simulink model "SwarmSystem"  (R2022b)
(part 3 of 4)

\"uuid\":\"66f2432a-d8da-4c77-847a-13be9309f023\"},{\"content\":{\"blockPath\":[\"SwarmSystem/Record\"],\"channel\":[7,2,1],\"dimensions\":[9,9,3],\"domain\":\"SwarmSystem/Record\",\"lineColor\":\"#ff6929\",\"parentID\":5326,\"plots\":[],\"port\":9,\"sid\":[\"\"],\"signalID\":5732,\"signalName\":\"packed_tw\"},\"type\":\"RecordBlkView.Signal\",\"uuid\":\"56f2028f-166f-4731-ad48-c59b44126da3\"},{\"content\":{\"blockPath\":[\"SwarmSystem/Record\"],\"channel\":[8,2,1],\"dimensions\":[9,9,3],\"domain\":\"SwarmSystem/Record\",\"lineColor\":\"#b746ff\",\"parentID\":5326,\"plots\":[],\"port\":9,\"sid\":[\"\"],\"signalID\":5733,\"signalName\":\"packed_tw\"},\"type\":\"RecordBlkView.Signal\",\"uuid\":\"6663be21-9b2e-46ef-97ca-d0d1a511769f\"},{\"content\":{\"blockPath\":[\"SwarmSystem/Record\"],\"channel\":[9,2,1],\"dimensions\":[9,9,3],\"domain\":\"SwarmSystem/Record\",\"lineColor\":\"#64d413\",\"parentID\":5326,\"plots\":[],\"port\":9,\"sid\":[\"\"],\"signalID\":5734,\"signalName\":\"packed_tw\"},\"type\":\"RecordBlkView.Signal\",\"uuid\":\"2c203f91-17b3-4c19-9696-d99f0a1ca0fd\"},{\"content\":{\"blockPath\":[\"SwarmSystem/Record\"],\"channel\":[1,3,1],\"dimensions\":[9,9,3],\"domain\":\"SwarmSystem/Record\",\"lineColor\":\"#ff13a6\",\"parentID\":5326,\"plots\":[],\"port\":9,\"sid\":[\"\"],\"signalID\":5735,\"signalName\":\"packed_tw\"},\"type\":\"RecordBlkView.Signal\",\"uuid\":\"a7da77ac-4730-4896-99b2-25e0e7a6f8af\"},{\"content\":{\"blockPath\":[\"SwarmSystem/Record\"],\"channel\":[2,3,1],\"dimensions\":[9,9,3],\"domain\":\"SwarmSystem/Record\",\"lineColor\":\"#fe330a\",\"parentID\":5326,\"plots\":[],\"port\":9,\"sid\":[\"\"],\"signalID\":5736,\"signalName\":\"packed_tw\"},\"type\":\"RecordBlkView.Signal\",\"uuid\":\"1e600a43-36ad-42ac-b351-5715d6370cc7\"},{\"content\":{\"blockPath\":[\"SwarmSystem/Record\"],\"channel\":[3,3,1],\"dimensions\":[9,9,3],\"domain\":\"SwarmSystem/Record\",\"lineColor\":\"#22b573\",\"parentID\":5326,\"plots\":[],\"port\":9,\"sid\":[\"\"],\"signalID\":5737,\"signalName\":\"packed_tw\"},\"type\":\"RecordBlkView.Signal\",\"uuid\":\"10fccabd-f891-426d-aafe-525a94df6eca\"},{\"content\":{\"blockPath\":[\"SwarmSystem/Record\"],\"channel\":[4,3,1],\"dimensions\":[9,9,3],\"domain\":\"SwarmSystem/Record\",\"lineColor\":\"#0072bd\",\"parentID\":5326,\"plots\":[],\"port\":9,\"sid\":[\"\"],\"signalID\":5738,\"signalName\":\"packed_tw\"},\"type\":\"RecordBlkView.Signal\",\"uuid\":\"d8f853b9-8d61-485c-b86b-01323a9b1dcc\"},{\"content\":{\"blockPath\":[\"SwarmSystem/Record\"],\"channel\":[5,3,1],\"dimensions\":[9,9,3],\"domain\":\"SwarmSystem/Record\",\"lineColor\":\"#d95319\",\"parentID\":5326,\"plots\":[],\"port\":9,\"sid\":[\"\"],\"signalID\":5739,\"signalName\":\"packed_tw\"},\"type\":\"RecordBlkView.Signal\",\"uuid\":\"32f64f79-0b5d-41ec-b8f2-db72d15c3b46\"},{\"content\":{\"blockPath\":[\"SwarmSystem/Record\"],\"channel\":[6,3,1],\"dimensions\":[9,9,3],\"domain\":\"SwarmSystem/Record\",\"lineColor\":\"#edb120\",\"parentID\":5326,\"plots\":[],\"port\":9,\"sid\":[\"\"],\"signalID\":5740,\"signalName\":\"packed_tw\"},\"type\":\"RecordBlkView.Signal\",\"uuid\":\"6bb0f485-e50d-4674-9966-5c0abecf3566\"},{\"content\":{\"blockPath\":[\"SwarmSystem/Record\"],\"channel\":[7,3,1],\"dimensions\":[9,9,3],\"domain\":\"SwarmSystem/Record\",\"lineColor\":\"#7e2f8e\",\"parentID\":5326,\"plots\":[],\"port\":9,\"sid\":[\"\"],\"signalID\":5741,\"signalName\":\"packed_tw\"},\"type\":\"RecordBlkView.Signal\",\"uuid\":\"efdbdfa0-ad42-48dc-a3e2-49e98de60d36\"},{\"content\":{\"blockPath\":[\"SwarmSystem/Record\"],\"channel\":[8,3,1],\"dimensions\":[9,9,3],\"domain\":\"SwarmSystem/Record\",\"lineColor\":\"#77ac30\",\"parentID\":5326,\"plots\":[],\"port\":9,\"sid\":[\"\"],\"signalID\":5742,\"signalName\":\"packed_tw\"},\"type\":\"RecordBlkView.Signal\",\"uuid\":\"b0fc06d3-33ee-41bb-9294-d6c8533c9df3\"},{\"content\":{\"blockPath\":[\"SwarmSystem/Record\"],\"channel\":[9,3,1],\"dimensions\":[9,9,3],\"domain\":\"SwarmSystem/Record\",\"lineColor\":\"#4dbeee\",\"parentID\":5326,\"plots\":[],\"port\":9,\"sid\":[\"\"],\"signalID\":5743,\"signalName\":\"packed_tw\"},\"type\":\"RecordBlkView.Signal\",\"uuid\":\"376f8440-522b-4ce7-8b3c-728053a193f3\"},{\"content\":{\"blockPath\":[\"SwarmSystem/Record\"],\"channel\":[1,4,1],\"dimensions\":[9,9,3],\"domain\":\"SwarmSystem/Record\",\"lineColor\":\"#a2142f\",\"parentID\":5326,\"plots\":[],\"port\":9,\"sid\":[\"\"],\"signalID\":5744,\"signalName\":\"packed_tw\"},\"type\":\"RecordBlkView.Signal\",\"uuid\":\"16833fa1-bc7e-4160-bf2a-8aa71fa237a6\"},{\"content\":{\"blockPath\":[\"SwarmSystem/Record\"],\"channel\":[2,4,1],\"dimensions\":[9,9,3],\"domain\":\"SwarmSystem/Record\",\"lineColor\":\"#139fff\",\"parentID\":5326,\"plots\":[],\"port\":9,\"sid\":[\"\"],\"signalID\":5745,\"signalName\":\"packed_tw\"},\"type\":\"RecordBlkView.Signal\",\"uuid\":\"0f9268d8-1260-481f-958d-5a37cc72ea48\"},{\"content\":{\"blockPath\":[\"SwarmSystem/Record\"],\"channel\":[3,4,1],\"dimensions\":[9,9,3],\"domain\":\"SwarmSystem/Record\",\"lineColor\":\"#ff6929\",\"parentID\":5326,\"plots\":[],\"port\":9,\"sid\":[\"\"],\"signalID\":5746,\"signalName\":\"packed_tw\"},\"type\":\"RecordBlkView.Signal\",\"uuid\":\"582107cd-b22c-4bf8-875e-6a25fbec9bc4\"},{\"content\":{\"blockPath\":[\"SwarmSystem/Record\"],\"channel\":[4,4,1],\"dimensions\":[9,9,3],\"domain\":\"SwarmSystem/Record\",\"lineColor\":\"#b746ff\",\"parentID\":5326,\"plots\":[],\"port\":9,\"sid\":[\"\"],\"signalID\":5747,\"signalName\":\"packed_tw\"},\"type\":\"RecordBlkView.Signal\",\"uuid\":\"86fb42d5-9bfb-4257-8da5-ea0cdfb8f8a8\"},{\"content\":{\"blockPath\":[\"SwarmSystem/Record\"],\"channel\":[5,4,1],\"dimensions\":[9,9,3],\"domain\":\"SwarmSystem/Record\",\"lineColor\":\"#64d413\",\"parentID\":5326,\"plots\":[],\"port\":9,\"sid\":[\"\"],\"signalID\":5748,\"signalName\":\"packed_tw\"},\"type\":\"RecordBlkView.Signal\",\"uuid\":\"152469c8-5e3d-42f9-b5e4-54b25046ce6a\"},{\"content\":{\"blockPath\":[\"SwarmSystem/Record\"],\"channel\":[6,4,1],\"dimensions\":[9,9,3],\"domain\":\"SwarmSystem/Record\",\"lineColor\":\"#ff13a6\",\"parentID\":5326,\"plots\":[],\"port\":9,\"sid\":[\"\"],\"signalID\":5749,\"signalName\":\"packed_tw\"},\"type\":\"RecordBlkView.Signal\",\"uuid\":\"f025a8fe-ae08-4e09-9d36-edd1af49b1c7\"},{\"content\":{\"blockPath\":[\"SwarmSystem/Record\"],\"channel\":[7,4,1],\"dimensions\":[9,9,3],\"domain\":\"SwarmSystem/Record\",\"lineColor\":\"#fe330a\",\"parentID\":5326,\"plots\":[],\"port\":9,\"sid\":[\"\"],\"signalID\":5750,\"signalName\":\"packed_tw\"},\"type\":\"RecordBlkView.Signal\",\"uuid\":\"d6d3dd3c-ecca-4921-b9f8-a246ee4cded9\"},{\"content\":{\"blockPath\":[\"SwarmSystem/Record\"],\"channel\":[8,4,1],\"dimensions\":[9,9,3],\"domain\":\"SwarmSystem/Record\",\"lineColor\":\"#22b573\",\"parentID\":5326,\"plots\":[],\"port\":9,\"sid\":[\"\"],\"signalID\":5751,\"signalName\":\"packed_tw\"},\"type\":\"RecordBlkView.Signal\",\"uuid\":\"cb92334f-db7b-47eb-97a9-d6af63c7032c\"},{\"content\":{\"blockPath\":[\"SwarmSystem/Record\"],\"channel\":[9,4,1],\"dimensions\":[9,9,3],\"domain\":\"SwarmSystem/Record\",\"lineColor\":\"#0072bd\",\"parentID\":5326,\"plots\":[],\"port\":9,\"sid\":[\"\"],\"signalID\":5752,\"signalName\":\"packed_tw\"},\"type\":\"RecordBlkView.Signal\",\"uuid\":\"410ffef6-764f-4449-b289-13b898e3b605\"},{\"content\":{\"blockPath\":[\"SwarmSystem/Record\"],\"channel\":[1,5,1],\"dimensions\":[9,9,3],\"domain\":\"SwarmSystem/Record\",\"lineColor\":\"#d95319\",\"parentID\":5326,\"plots\":[],\"port\":9,\"sid\":[\"\"],\"signalID\":5753,\"signalName\":\"packed_tw\"},\"type\":\"RecordBlkView.Signal\",\"uuid\":\"e261075f-568b-4d5f-8c86-3e293640aaf6\"},{\"content\":{\"blockPath\":[\"SwarmSystem/Record\"],\"channel\":[2,5,1],\"dimensions\":[9,9,3],\"domain\":\"SwarmSystem/Record\",\"lineColor\":\"#edb120\",\"parentID\":5326,\"plots\":[],\"port\":9,\"sid\":[\"\"],\"signalID\":5754,\"signalName\":\"packed_tw\"},\"type\":\"RecordBlkView.Signal\",\"uuid\":\"02d9d080-5992-4875-a7e4-490970fd0aba\"},{\"content\":{\"blockPath\":[\"SwarmSystem/Record\"],\"channel\":[3,5,1],\"dimensions\":[9,9,3],\"domain\":\"SwarmSystem/Record\",\"lineColor\":\"#7e2f8e\",\"parentID\":5326,\"plots\":[],\"port\":9,\"sid\":[\"\"],\"signalID\":5755,\"signalName\":\"packed_tw\"},\"type\":\"RecordBlkView.Signal\",\"uuid\":\"f6234f5e-dfa5-4099-ab9d-213a77899b41\"},{\"content\":{\"blockPath\":[\"SwarmSystem/Record\"],\"channel\":[4,5,1],\"dimensions\":[9,9,3],\"domain\":\"SwarmSystem/Record\",\"lineColor\":\"#77ac30\",\"parentID\":5326,\"plots\":[],\"port\":9,\"sid\":[\"\"],\"signalID\":5756,\"signalName\":\"packed_tw\"},\"type\":\"RecordBlkView.Signal\",\"uuid\":\"897adc16-ad91-416a-abb4-75db18956903\"},{\"content\":{\"blockPath\":[\"SwarmSystem/Record\"],\"channel\":[5,5,1],\"dimensions\":[9,9,3],\"domain\":\"SwarmSystem/Record\",\"lineColor\":\"#4dbeee\",\"parentID\":5326,\"plots\":[],\"port\":9,\"sid\":[\"\"],\"signalID\":5757,\"signalName\":\"packed_tw\"},\"type\":\"RecordBlkView.Signal\",\"uuid\":\"0cc5aa6a-a08c-40bc-a91d-690ed3804433\"},{\"content\":{\"blockPath\":[\"SwarmSystem/Record\"],\"channel\":[6,5,1],\"dimensions\":[9,9,3],\"domain\":\"SwarmSystem/Record\",\"lineColor\":\"#a2142f\",\"parentID\":5326,\"plots\":[],\"port\":9,\"sid\":[\"\"],\"signalID\":5758,\"signalName\":\"packed_tw\"},\"type\":\"RecordBlkView.Signal\",\"uuid\":\"667ed152-3318-44bb-b581-6255efbc3158\"},{\"content\":{\"blockPath\":[\"SwarmSystem/Record\"],\"channel\":[7,5,1],\"dimensions\":[9,9,3],\"domain\":\"SwarmSystem/Record\",\"lineColor\":\"#139fff\",\"parentID\":5326,\"plots\":[],\"port\":9,\"sid\":[\"\"],\"signalID\":5759,\"signalName\":\"packed_tw\"},\"type\":\"RecordBlkView.Signal\",\"uuid\":\"c45443c0-bb0f-43ce-ae46-f6908f651d0a\"},{\"content\":{\"blockPath\":[\"SwarmSystem/Record\"],\"channel\":[8,5,1],\"dimensions\":[9,9,3],\"domain\":\"SwarmSystem/Record\",\"lineColor\":\"#ff6929\",\"parentID\":5326,\"plots\":[],\"port\":9,\"sid\":[\"\"],\"signalID\":5760,\"signalName\":\"packed_tw\"},\"type\":\"RecordBlkView.Signal\",\"uuid\":\"3b7accaa-1a50-42c4-810c-86a74667a25e\"},{\"content\":{\"blockPath\":[\"SwarmSystem/Record\"],\"channel\":[9,5,1],\"dimensions\":[9,9,3],\"domain\":\"SwarmSystem/Record\",\"lineColor\":\"#b746ff\",\"parentID\":5326,\"plots\":[],\"port\":9,\"sid\":[\"\"],\"signalID\":5761,\"signalName\":\"packed_tw\"},\"type\":\"RecordBlkView.Signal\",\"uuid\":\"4a9e9fa2-2054-41d9-b7b8-434b94a0f53e\"},{\"content\":{\"blockPath\":[\"SwarmSystem/Record\"],\"channel\":[1,6,1],\"dimensions\":[9,9,3],\"domain\":\"SwarmSystem/Record\",\"lineColor\":\"#64d413\",\"parentID\":5326,\"plots\":[],\"port\":9,\"sid\":[\"\"],\"signalID\":5762,\"signalName\":\"packed_tw\"},\"type\":\"RecordBlkView.Signal\",\"uuid\":\"2f297c1c-5db3-4597-bca3-5568c9b68469\"},{\"content\":{\"blockPath\":[\"SwarmSystem/Record\"],\"channel\":[2,6,1],\"dimensions\":[9,9,3],\"domain\":\"SwarmSystem/Record\",\"lineColor\":\"#ff13a6\",\"parentID\":5326,\"plots\":[],\"port\":9,\"sid\":[\"\"],\"signalID\":5763,\"signalName\":\"packed_tw\"},\"type\":\"RecordBlkView.Signal\",\"uuid\":\"3bcefa39-97a0-4915-bf31-1d3eb75403ff\"},{\"content\":{\"blockPath\":[\"SwarmSystem/Record\"],\"channel\":[3,6,1],\"dimensions\":[9,9,3],\"domain\":\"SwarmSystem/Record\",\"lineColor\":\"#fe330a\",\"parentID\":5326,\"plots\":[],\"port\":9,\"sid\":[\"\"],\"signalID\":5764,\"signalName\":\"packed_tw\"},\"type\":\"RecordBlkView.Signal\",\"uuid\":\"26a823e5-a67c-4fe0-8814-e404e1866f34\"},{\"content\":{\"blockPath\":[\"SwarmSystem/Record\"],\"channel\":[4,6,1],\"dimensions\":[9,9,3],\"domain\":\"SwarmSystem/Record\",\"lineColor\":\"#22b573\",\"parentID\":5326,\"plots\":[],\"port\":9,\"sid\":[\"\"],\"signalID\":5765,\"signalName\":\"packed_tw\"},\"type\":\"RecordBlkView.Signal\",\"uuid\":\"0219ef0b-387c-40a0-97df-a2f3b60856a0\"},{\"content\":{\"blockPath\":[\"SwarmSystem/Record\"],\"channel\":[5,6,1],\"dimensions\":[9,9,3],\"domain\":\"SwarmSystem/Record\",\"lineColor\":\"#0072bd\",\"parentID\":5326,\"plots\":[],\"port\":9,\"sid\":[\"\"],\"signalID\":5766,\"signalName\":\"packed_tw\"},\"type\":\"RecordBlkView.Signal\",\"uuid\":\"e0fe79da-d3e3-475c-af43-7a4fae6dd308\"},{\"content\":{\"blockPath\":[\"SwarmSystem/Record\"],\"channel\":[6,6,1],\"dimensions\":[9,9,3],\"domain\":\"SwarmSystem/Record\",\"lineColor\":\"#d95319\",\"parentID\":5326,\"plots\":[],\"port\":9,\"sid\":[\"\"],\"signalID\":5767,\"signalName\":\"packed_tw\"},\"type\":\"RecordBlkView.Signal\",\"uuid\":\"25247346-aef6-4321-9915-4b5ba2b68a3c\"},{\"content\":{\"blockPath\":[\"SwarmSystem/Record\"],\"channel\":[7,6,1],\"dimensions\":[9,9,3],\"domain\":\"SwarmSystem/Record\",\"lineColor\":\"#edb120\",\"parentID\":5326,\"plots\":[],\"port\":9,\"sid\":[\"\"],\"signalID\":5768,\"signalName\":\"packed_tw\"},\"type\":\"RecordBlkView.Signal\",\"uuid\":\"d5d8b9f2-a0d1-4825-ac7f-db45dff184b1\"},{\"content\":{\"blockPath\":[\"SwarmSystem/Record\"],\"channel\":[8,6,1],\"dimensions\":[9,9,3],\"domain\":\"SwarmSystem/Record\",\"lineColor\":\"#7e2f8e\",\"parentID\":5326,\"plots\":[],\"port\":9,\"sid\":[\"\"],\"signalID\":5769,\"signalName\":\"packed_tw\"},\"type\":\"RecordBlkView.Signal\",\"uuid\":\"c3c3fecf-6756-4264-a6b3-b17d8feaae56\"},{\"content\":{\"blockPath\":[\"SwarmSystem/Record\"],\"channel\":[9,6,1],\"dimensions\":[9,9,3],\"domain\":\"SwarmSystem/Record\",\"lineColor\":\"#77ac30\",\"parentID\":5326,\"plots\":[],\"port\":9,\"sid\":[\"\"],\"signalID\":5770,\"signalName\":\"packed_tw\"},\"type\":\"RecordBlkView.Signal\",\"uuid\":\"95d6af73-0c27-4f58-aa73-e4afb520c9b6\"},{\"content\":{\"blockPath\":[\"SwarmSystem/Record\"],\"channel\":[1,7,1],\"dimensions\":[9,9,3],\"domain\":\"SwarmSystem/Record\",\"lineColor\":\"#4dbeee\",\"parentID\":5326,\"plots\":[],\"port\":9,\"sid\":[\"\"],\"signalID\":5771,\"signalName\":\"packed_tw\"},\"type\":\"RecordBlkView.Signal\",\"uuid\":\"ffa40b6e-c93c-45e7-a825-7543730c02a7\"},{\"content\":{\"blockPath\":[\"SwarmSystem/Record\"],\"channel\":[2,7,1],\"dimensions\":[9,9,3],\"domain\":\"SwarmSystem/Record\",\"lineColor\":\"#a2142f\",\"parentID\":5326,\"plots\":[],\"port\":9,\"sid\":[\"\"],\"signalID\":5772,\"signalName\":\"packed_tw\"},\"type\":\"RecordBlkView.Signal\",\"uuid\":\"572a2db8-4bea-405f-acfc-7af25e433108\"},{\"content\":{\"blockPath\":[\"SwarmSystem/Record\"],\"channel\":[3,7,1],\"dimensions\":[9,9,3],\"domain\":\"SwarmSystem/Record\",\"lineColor\":\"#139fff\",\"parentID\":5326,\"plots\":[],\"port\":9,\"sid\":[\"\"],\"signalID\":5773,\"signalName\":\"packed_tw\"},\"type\":\"RecordBlkView.Signal\",\"uuid\":\"0dfc27a1-e3b2-4639-b1fe-a522ef6232c5\"},{\"content\":{\"blockPath\":[\"SwarmSystem/Record\"],\"channel\":[4,7,1],\"dimensions\":[9,9,3],\"domain\":\"SwarmSystem/Record\",\"lineColor\":\"#ff6929\",\"parentID\":5326,\"plots\":[],\"port\":9,\"sid\":[\"\"],\"signalID\":5774,\"signalName\":\"packed_tw\"},\"type\":\"RecordBlkView.Signal\",\"uuid\":\"6f7742b4-e30b-4d3b-9c5b-bb79d8c25ffc\"},{\"content\":{\"blockPath\":[\"SwarmSystem/Record\"],\"channel\":[5,7,1],\"dimensions\":[9,9,3],\"domain\":\"SwarmSystem/Record\",\"lineColor\":\"#b746ff\",\"parentID\":5326,\"plots\":[],\"port\":9,\"sid\":[\"\"],\"signalID\":5775,\"signalName\":\"packed_tw\"},\"type\":\"RecordBlkView.Signal\",\"uuid\":\"1bed10ed-21c7-4778-9f87-780cf6804573\"},{\"content\":{\"blockPath\":[\"SwarmSystem/Record\"],\"channel\":[6,7,1],\"dimensions\":[9,9,3],\"domain\":\"SwarmSystem/Record\",\"lineColor\":\"#64d413\",\"parentID\":5326,\"plots\":[],\"port\":9,\"sid\":[\"\"],\"signalID\":5776,\"signalName\":\"packed_tw\"},\"type\":\"RecordBlkView.Signal\",\"uuid\":\"f026d189-9db8-4d86-976b-f51f0daa1cbb\"},{\"content\":{\"blockPath\":[\"SwarmSystem/Record\"],\"channel\":[7,7,1],\"dimensions\":[9,9,3],\"domain\":\"SwarmSystem/Record\",\"lineColor\":\"#ff13a6\",\"parentID\":5326,\"plots\":[],\"port\":9,\"sid\":[\"\"],\"signalID\":5777,\"signalName\":\"packed_tw\"},\"type\":\"RecordBlkView.Signal\",\"uuid\":\"693525ca-a567-456e-a572-dbfb87322e0c\"},{\"content\":{\"blockPath\":[\"SwarmSystem/Record\"],\"channel\":[8,7,1],\"dimensions\":[9,9,3],\"domain\":\"SwarmSystem/Record\",\"lineColor\":\"#fe330a\",\"parentID\":5326,\"plots\":[],\"port\":9,\"sid\":[\"\"],\"signalID\":5778,\"signalName\":\"packed_tw\"},\"type\":\"RecordBlkView.Signal\",\"uuid\":\"67c23147-ccbd-4398-b187-1940e8bea18b\"},{\"content\":{\"blockPath\":[\"SwarmSystem/Record\"],\"channel\":[9,7,1],\"dimensions\":[9,9,3],\"domain\":\"SwarmSystem/Record\",\"lineColor\":\"#22b573\",\"parentID\":5326,\"plots\":[],\"port\":9,\"sid\":[\"\"],\"signalID\":5779,\"signalName\":\"packed_tw\"},\"type\":\"RecordBlkView.Signal\",\"uuid\":\"97770466-2798-420b-969b-754700610d6d\"},{\"content\":{\"blockPath\":[\"SwarmSystem/Record\"],\"channel\":[1,8,1],\"dimensions\":[9,9,3],\"domain\":\"SwarmSystem/Record\",\"lineColor\":\"#0072bd\",\"parentID\":5326,\"plots\":[],\"port\":9,\"sid\":[\"\"],\"signalID\":5780,\"signalName\":\"packed_tw\"},\"type\":\"RecordBlkView.Signal\",\"uuid\":\"c0d727bd-d530-42f1-bdd3-579b10f7c70f\"},{\"content\":{\"blockPath\":[\"SwarmSystem/Record\"],\"channel\":[2,8,1],\"dimensions\":[9,9,3],\"domain\":\"SwarmSystem/Record\",\"lineColor\":\"#d95319\",\"parentID\":5326,\"plots\":[],\"port\":9,\"sid\":[\"\"],\"signalID\":5781,\"signalName\":\"packed_tw\"},\"type\":\"RecordBlkView.Signal\",\"uuid\":\"e95a2d2e-be99-4a14-8ecc-e91ebfb0d15f\"},{\"content\":{\"blockPath\":[\"SwarmSystem/Record\"],\"channel\":[3,8,1],\"dimensions\":[9,9,3],\"domain\":\"SwarmSystem/Record\",\"lineColor\":\"#edb120\",\"parentID\":5326,\"plots\":[],\"port\":9,\"sid\":[\"\"],\"signalID\":5782,\"signalName\":\"packed_tw\"},\"type\":\"RecordBlkView.Signal\",\"uuid\":\"618e1a82-3965-4102-97cc-7656c92e492e\"},{\"content\":{\"blockPath\":[\"SwarmSystem/Record\"],\"channel\":[4,8,1],\"dimensions\":[9,9,3],\"domain\":\"SwarmSystem/Record\",\"lineColor\":\"#7e2f8e\",\"parentID\":5326,\"plots\":[],\"port\":9,\"sid\":[\"\"],\"signalID\":5783,\"signalName\":\"packed_tw\"},\"type\":\"RecordBlkView.Signal\",\"uuid\":\"5a512c5a-af72-415b-bdc8-3aa69033ccbb\"},{\"content\":{\"blockPath\":[\"SwarmSystem/Record\"],\"channel\":[5,8,1],\"dimensions\":[9,9,3],\"domain\":\"SwarmSystem/Record\",\"lineColor\":\"#77ac30\",\"parentID\":5326,\"plots\":[],\"port\":9,\"sid\":[\"\"],\"signalID\":5784,\"signalName\":\"packed_tw\"},\"type\":\"RecordBlkView.Signal\",\"uuid\":\"e955dfcf-7950-4eba-bd26-624af6308b70\"},{\"content\":{\"blockPath\":[\"SwarmSystem/Record\"],\"channel\":[6,8,1],\"dimensions\":[9,9,3],\"domain\":\"SwarmSystem/Record\",\"lineColor\":\"#4dbeee\",\"parentID\":5326,\"plots\":[],\"port\":9,\"sid\":[\"\"],\"signalID\":5785,\"signalName\":\"packed_tw\"},\"type\":\"RecordBlkView.Signal\",\"uuid\":\"ece48233-0de4-42a5-9ae6-f029001ff023\"},{\"content\":{\"blockPath\":[\"SwarmSystem/Record\"],\"channel\":[7,8,1],\"dimensions\":[9,9,3],\"domain\":\"SwarmSystem/Record\",\"lineColor\":\"#a2142f\",\"parentID\":5326,\"plots\":[],\"port\":9,\"sid\":[\"\"],\"signalID\":5786,\"signalName\":\"packed_tw\"},\"type\":\"RecordBlkView.Signal\",\"uuid\":\"824bdf22-e070-493b-b58d-fb5a60069d4e\"},{\"content\":{\"blockPath\":[\"SwarmSystem/Record\"],\"channel\":[8,8,1],\"dimensions\":[9,9,3],\"domain\":\"SwarmSystem/Record\",\"lineColor\":\"#139fff\",\"parentID\":5326,\"plots\":[],\"port\":9,\"sid\":[\"\"],\"signalID\":5787,\"signalName\":\"packed_tw\"},\"type\":\"RecordBlkView.Signal\",\"uuid\":\"caa1d600-3dac-4235-a1df-80f1f38b6da0\"},{\"content\":{\"blockPath\":[\"SwarmSystem/Record\"],\"channel\":[9,8,1],\"dimensions\":[9,9,3],\"domain\":\"SwarmSystem/Record\",\"lineColor\":\"#ff6929\",\"parentID\":5326,\"plots\":[],\"port\":9,\"sid\":[\"\"],\"signalID\":5788,\"signalName\":\"packed_tw\"},\"type\":\"RecordBlkView.Signal\",\"uuid\":\"70268a07-477f-46a3-bb7c-da2b62262bc9\"},{\"content\":{\"blockPath\":[\"SwarmSystem/Record\"],\"channel\":[1,9,1],\"dimensions\":[9,9,3],\"domain\":\"SwarmSystem/Record\",\"lineColor\":\"#b746ff\",\"parentID\":5326,\"plots\":[],\"port\":9,\"sid\":[\"\"],\"signalID\":5789,\"signalName\":\"packed_tw\"},\"type\":\"RecordBlkView.Signal\",\"uuid\":\"d68f7306-5943-43c0-978b-d9ecc93acb51\"},{\"content\":{\"blockPath\":[\"SwarmSystem/Record\"],\"channel\":[2,9,1],\"dimensions\":[9,9,3],\"domain\":\"SwarmSystem/Record\",\"lineColor\":\"#64d413\",\"parentID\":5326,\"plots\":[],\"port\":9,\"sid\":[\"\"],\"signalID\":5790,\"signalName\":\"packed_tw\"},\"type\":\"RecordBlkView.Signal\",\"uuid\":\"edf609c4-3d89-44f9-9262-dda908b0e004\"},{\"content\":{\"blockPath\":[\"SwarmSystem/Record\"],\"channel\":[3,9,1],\"dimensions\":[9,9,3],\"domain\":\"SwarmSystem/Record\",\"lineColor\":\"#ff13a6\",\"parentID\":5326,\"plots\":[],\"port\":9,\"sid\":[\"\"],\"signalID\":5791,\"signalName\":\"packed_tw\"},\"type\":\"RecordBlkView.Signal\",\"uuid\":\"1f514293-d0a4-426d-8fe5-839bc86e8e90\"},{\"content\":{\"blockPath\":[\"SwarmSystem/Record\"],\"channel\":[4,9,1],\"dimensions\":[9,9,3],\"domain\":\"SwarmSystem/Record\",\"lineColor\":\"#fe330a\",\"parentID\":5326,\"plots\":[],\"port\":9,\"sid\":[\"\"],\"signalID\":5792,\"signalName\":\"packed_tw\"},\"type\":\"RecordBlkView.Signal\",\"uuid\":\"9ed22710-5236-4372-8da5-48d9aff1790b\"},{\"content\":{\"blockPath\":[\"SwarmSystem/Record\"],\"channel\":[5,9,1],\"dimensions\":[9,9,3],\"domain\":\"SwarmSystem/Record\",\"lineColor\":\"#22b573\",\"parentID\":5326,\"plots\":[],\"port\":9,\"sid\":[\"\"],\"signalID\":5793,\"signalName\":\"packed_tw\"},\"type\":\"RecordBlkView.Signal\",\"uuid\":\"31fcf3e9-d45c-439a-97b6-eb5fde562b10\"},{\"content\":{\"blockPath\":[\"SwarmSystem/Record\"],\"channel\":[6,9,1],\"dimensions\":[9,9,3],\"domain\":\"SwarmSystem/Record\",\"lineColor\":\"#0072bd\",\"parentID\":5326,\"plots\":[],\"port\":9,\"sid\":[\"\"],\"signalID\":5794,\"signalName\":\"packed_tw\"},\"type\":\"RecordBlkView.Signal\",\"uuid\":\"9bcc6742-29be-48e2-89c3-fd54e1edf038\"},{\"content\":{\"blockPath\":[\"SwarmSystem/Record\"],\"channel\":[7,9,1],\"dimensions\":[9,9,3],\"domain\":\"SwarmSystem/Record\",\"lineColor\":\"#d95319\",\"parentID\":5326,\"plots\":[],\"port\":9,\"sid\":[\"\"],\"signalID\":5795,\"signalName\":\"packed_tw\"},\"type\":\"RecordBlkView.Signal\",\"uuid\":\"961200f8-714d-4018-af6a-2f1112332411\"},{\"content\":{\"blockPath\":[\"SwarmSystem/Record\"],\"channel\":[8,9,1],\"dimensions\":[9,9,3],\"domain\":\"SwarmSystem/Record\",\"lineColor\":\"#edb120\",\"parentID\":5326,\"plots\":[],\"port\":9,\"sid\":[\"\"],\"signalID\":5796,\"signalName\":\"packed_tw\"},\"type\":\"RecordBlkView.Signal\",\"uuid\":\"c1ea7ad4-a570-4cc9-90b0-014c375aaef8\"},{\"content\":{\"blockPath\":[\"SwarmSystem/Record\"],\"channel\":[9,9,1],\"dimensions\":[9,9,3],\"domain\":\"SwarmSystem/Record\",\"lineColor\":\"#7e2f8e\",\"parentID\":5326,\"plots\":[],\"port\":9,\"sid\":[\"\"],\"signalID\":5797,\"signalName\":\"packed_tw\"},\"type\":\"RecordBlkView.Signal\",\"uuid\":\"cb727bd5-f244-448c-a21d-edf04e397600\"},{\"content\":{\"blockPath\":[\"SwarmSystem/Record\"],\"channel\":[1,1,2],\"dimensions\":[9,9,3],\"domain\":\"SwarmSystem/Record\",\"lineColor\":\"#77ac30\",\"parentID\":5326,\"plots\":[],\"port\":9,\"sid\":[\"\"],\"signalID\":5798,\"signalName\":\"packed_tw\"},\"type\":\"RecordBlkView.Signal\",\"uuid\":\"cb38d9e5-ffd7-459c-8e44-38c3f8cd33c6\"},{\"content\":{\"blockPath\":[\"SwarmSystem/Record\"],\"channel\":[2,1,2],\"dimensions\":[9,9,3],\"domain\":\"SwarmSystem/Record\",\"lineColor\":\"#4dbeee\",\"parentID\":5326,\"plots\":[],\"port\":9,\"sid\":[\"\"],\"signalID\":5799,\"signalName\":\"packed_tw\"},\"type\":\"RecordBlkView.Signal\",\"uuid\":\"25e48605-b9a0-4eff-9681-4ea1dedc7113\"},{\"content\":{\"blockPath\":[\"SwarmSystem/Record\"],\"channel\":[3,1,2],\"dimensions\":[9,9,3],\"domain\":\"SwarmSystem/Record\",\"lineColor\":\"#a2142f\",\"parentID\":5326,\"plots\":[],\"port\":9,\"sid\":[\"\"],\"signalID\":5800,\"signalName\":\"packed_tw\"},\"type\":\"RecordBlkView.Signal\",\"uuid\":\"46ac54a4-10b4-4c2f-a611-f8be5c9883b4\"},{\"content\":{\"blockPath\":[\"SwarmSystem/Record\"],\"channel\":[4,1,2],\"dimensions\":[9,9,3],\"domain\":\"SwarmSystem/Record\",\"lineColor\":\"#139fff\",\"parentID\":5326,\"plots\":[],\"port\":9,\"sid\":[\"\"],\"signalID\":5801,\"signalName\":\"packed_tw\"},\"type\":\"RecordBlkView.Signal\",\"uuid\":\"ac218199-2d6d-4ea5-a8c1-aacdddd33c28\"},{\"content\":{\"blockPath\":[\"SwarmSystem/Record\"],\"channel\":[5,1,2],\"dimensions\":[9,9,3],\"domain\":\"SwarmSystem/Record\",\"lineColor\":\"#ff6929\",\"parentID\":5326,\"plots\":[],\"port\":9,\"sid\":[\"\"],\"signalID\":5802,\"signalName\":\"packed_tw\"},\"type\":\"RecordBlkView.Signal\",\"uuid\":\"f55d1ba3-9854-45c1-8251-dd3b01695bb6\"},{\"content\":{\"blockPath\":[\"SwarmSystem/Record\"],\"channel\":[6,1,2],\"dimensions\":[9,9,3],\"domain\":\"SwarmSystem/Record\",\"lineColor\":\"#b746ff\",\"parentID\":5326,\"plots\":[],\"port\":9,\"sid\":[\"\"],\"signalID\":5803,\"signalName\":\"packed_tw\"},\"type\":\"RecordBlkView.Signal\",\"uuid\":\"024d7ef1-8905-4559-97f9-831c79e47f0f\"},{\"content\":{\"blockPath\":[\"SwarmSystem/Record\"],\"channel\":[7,1,2],\"dimensions\":[9,9,3],\"domain\":\"SwarmSystem/Record\",\"lineColor\":\"#64d413\",\"parentID\":5326,\"plots\":[],\"port\":9,\"sid\":[\"\"],\"signalID\":5804,\"signalName\":\"packed_tw\"},\"type\":\"RecordBlkView.Signal\",\"uuid\":\"8ccd5203-03c3-4fcd-94b7-203d27d26910\"},{\"content\":{\"blockPath\":[\"SwarmSystem/Record\"],\"channel\":[8,1,2],\"dimensions\":[9,9,3],\"domain\":\"SwarmSystem/Record\",\"lineColor\":\"#ff13a6\",\"parentID\":5326,\"plots\":[],\"port\":9,\"sid\":[\"\"],\"signalID\":5805,\"signalName\":\"packed_tw\"},\"type\":\"RecordBlkView.Signal\",\"uuid\":\"6dd5faa0-5582-4c32-84a6-9e6d74d4ab74\"},{\"content\":{\"blockPath\":[\"SwarmSystem/Record\"],\"channel\":[9,1,2],\"dimensions\":[9,9,3],\"domain\":\"SwarmSystem/Record\",\"lineColor\":\"#fe330a\",\"parentID\":5326,\"plots\":[],\"port\":9,\"sid\":[\"\"],\"signalID\":5806,\"signalName\":\"packed_tw\"},\"type\":\"RecordBlkView.Signal\",\"uuid\":\"effa1f6f-5389-411d-88e5-57b121372908\"},{\"content\":{\"blockPath\":[\"SwarmSystem/Record\"],\"channel\":[1,2,2],\"dimensions\":[9,9,3],\"domain\":\"SwarmSystem/Record\",\"lineColor\":\"#22b573\",\"parentID\":5326,\"plots\":[],\"port\":9,\"sid\":[\"\"],\"signalID\":5807,\"signalName\":\"packed_tw\"},\"type\":\"RecordBlkView.Signal\",\"uuid\":\"60e694a9-3551-482f-9541-9e908d86fb43\"},{\"content\":{\"blockPath\":[\"SwarmSystem/Record\"],\"channel\":[2,2,2],\"dimensions\":[9,9,3],\"domain\":\"SwarmSystem/Record\",\"lineColor\":\"#0072bd\",\"parentID\":5326,\"plots\":[],\"port\":9,\"sid\":[\"\"],\"signalID\":5808,\"signalName\":\"packed_tw\"},\"type\":\"RecordBlkView.Signal\",\"uuid\":\"64585b29-3283-4af9-89d1-c59c492422c2\"},{\"content\":{\"blockPath\":[\"SwarmSystem/Record\"],\"channel\":[3,2,2],\"dimensions\":[9,9,3],\"domain\":\"SwarmSystem/Record\",\"lineColor\":\"#d95319\",\"parentID\":5326,\"plots\":[],\"port\":9,\"sid\":[\"\"],\"signalID\":5809,\"signalName\":\"packed_tw\"},\"type\":\"RecordBlkView.Signal\",\"uuid\":\"e1f20fe9-1db5-4066-87d6-318fe0e498e9\"},{\"content\":{\"blockPath\":[\"SwarmSystem/Record\"],\"channel\":[4,2,2],\"dimensions\":[9,9,3],\"domain\":\"SwarmSystem/Record\",\"lineColor\":\"#edb120\",\"parentID\":5326,\"plots\":[],\"port\":9,\"sid\":[\"\"],\"signalID\":5810,\"signalName\":\"packed_tw\"},\"type\":\"RecordBlkView.Signal\",\"uuid\":\"930acee9-4257-4c9a-99a8-349e59c5c7d9\"},{\"content\":{\"blockPath\":[\"SwarmSystem/Record\"],\"channel\":[5,2,2],\"dimensions\":[9,9,3],\"domain\":\"SwarmSystem/Record\",\"lineColor\":\"#7e2f8e\",\"parentID\":5326,\"plots\":[],\"port\":9,\"sid\":[\"\"],\"signalID\":5811,\"signalName\":\"packed_tw\"},\"type\":\"RecordBlkView.Signal\",\"uuid\":\"42f198cf-b7e2-45a5-8eec-73d355926375\"},{\"content\":{\"blockPath\":[\"SwarmSystem/Record\"],\"channel\":[6,2,2],\"dimensions\":[9,9,3],\"domain\":\"SwarmSystem/Record\",\"lineColor\":\"#77ac30\",\"parentID\":5326,\"plots\":[],\"port\":9,\"sid\":[\"\"],\"signalID\":5812,\"signalName\":\"packed_tw\"},\"type\":\"RecordBlkView.Signal\",\"uuid\":\"af41296c-0c3d-45c8-a859-59d45e13e9c2\"},{\"content\":{\"blockPath\":[\"SwarmSystem/Record\"],\"channel\":[7,2,2],\"dimensions\":[9,9,3],\"domain\":\"SwarmSystem/Record\",\"lineColor\":\"#4dbeee\",\"parentID\":5326,\"plots\":[],\"port\":9,\"sid\":[\"\"],\"signalID\":5813,\"signalName\":\"packed_tw\"},\"type\":\"RecordBlkView.Signal\",\"uuid\":\"e673c85c-3b38-4b09-a889-1e246211c421\"},{\"content\":{\"blockPath\":[\"SwarmSystem/Record\"],\"channel\":[8,2,2],\"dimensions\":[9,9,3],\"domain\":\"SwarmSystem/Record\",\"lineColor\":\"#a2142f\",\"parentID\":5326,\"plots\":[],\"port\":9,\"sid\":[\"\"],\"signalID\":5814,\"signalName\":\"packed_tw\"},\"type\":\"RecordBlkView.Signal\",\"uuid\":\"0ef2cfa8-3698-4975-baf2-f02ae27c6b5c\"},{\"content\":{\"blockPath\":[\"SwarmSystem/Record\"],\"channel\":[9,2,2],\"dimensions\":[9,9,3],\"domain\":\"SwarmSystem/Record\",\"lineColor\":\"#139fff\",\"parentID\":5326,\"plots\":[],\"port\":9,\"sid\":[\"\"],\"signalID\":5815,\"signalName\":\"packed_tw\"},\"type\":\"RecordBlkView.Signal\",\"uuid\":\"2c305bdd-f00d-47e3-a104-3da68df50175\"},{\"content\":{\"blockPath\":[\"SwarmSystem/Record\"],\"channel\":[1,3,2],\"dimensions\":[9,9,3],\"domain\":\"SwarmSystem/Record\",\"lineColor\":\"#ff6929\",\"parentID\":5326,\"plots\":[],\"port\":9,\"sid\":[\"\"],\"signalID\":5816,\"signalName\":\"packed_tw\"},\"type\":\"RecordBlkView.Signal\",\"uuid\":\"553ce6f2-2ed6-40c5-a20e-983dfc431183\"},{\"content\":{\"blockPath\":[\"SwarmSystem/Record\"],\"channel\":[2,3,2],\"dimensions\":[9,9,3],\"domain\":\"SwarmSystem/Record\",\"lineColor\":\"#b746ff\",\"parentID\":5326,\"plots\":[],\"port\":9,\"sid\":[\"\"],\"signalID\":5817,\"signalName\":\"packed_tw\"},\"type\":\"RecordBlkView.Signal\",\"uuid\":\"89f353a5-7a81-461b-a22e-736f12088d8e\"},{\"content\":{\"blockPath\":[\"SwarmSystem/Record\"],\"channel\":[3,3,2],\"dimensions\":[9,9,3],\"domain\":\"SwarmSystem/Record\",\"lineColor\":\"#64d413\",\"parentID\":5326,\"plots\":[],\"port\":9,\"sid\":[\"\"],\"signalID\":5818,\"signalName\":\"packed_tw\"},\"type\":\"RecordBlkView.Signal\",\"uuid\":\"9c8ba869-9418-4a08-8767-18862245c084\"},{\"content\":{\"blockPath\":[\"SwarmSystem/Record\"],\"channel\":[4,3,2],\"dimensions\":[9,9,3],\"domain\":\"SwarmSystem/Record\",\"lineColor\":\"#ff13a6\",\"parentID\":5326,\"plots\":[],\"port\":9,\"sid\":[\"\"],\"signalID\":5819,\"signalName\":\"packed_tw\"},\"type\":\"RecordBlkView.Signal\",\"uuid\":\"c861881c-da11-4fd0-b8fb-73a7150c480e\"},{\"content\":{\"blockPath\":[\"SwarmSystem/Record\"],\"channel\":[5,3,2],\"dimensions\":[9,9,3],\"domain\":\"SwarmSystem/Record\",\"lineColor\":\"#fe330a\",\"parentID\":5326,\"plots\":[],\"port\":9,\"sid\":[\"\"],\"signalID\":5820,\"signalName\":\"packed_tw\"},\"type\":\"RecordBlkView.Signal\",\"uuid\":\"c9f9dad2-6c58-4512-ba52-96053e8c0cac\"},{\"content\":{\"blockPath\":[\"SwarmSystem/Record\"],\"channel\":[6,3,2],\"dimensions\":[9,9,3],\"domain\":\"SwarmSystem/Record\",\"lineColor\":\"#22b573\",\"parentID\":5326,\"plots\":[],\"port\":9,\"sid\":[\"\"],\"signalID\":5821,\"signalName\":\"packed_tw\"},\"type\":\"RecordBlkView.Signal\",\"uuid\":\"316f2dc2-43f8-48d7-88b4-a124a1a2146f\"},{\"content\":{\"blockPath\":[\"SwarmSystem/Record\"],\"channel\":[7,3,2],\"dimensions\":[9,9,3],\"domain\":\"SwarmSystem/Record\",\"lineColor\":\"#0072bd\",\"parentID\":5326,\"plots\":[],\"port\":9,\"sid\":[\"\"],\"signalID\":5822,\"signalName\":\"packed_tw\"},\"type\":\"RecordBlkView.Signal\",\"uuid\":\"00eb1436-1d6d-4b52-8758-987c3d3c700f\"},{\"content\":{\"blockPath\":[\"SwarmSystem/Record\"],\"channel\":[8,3,2],\"dimensions\":[9,9,3],\"domain\":\"SwarmSystem/Record\",\"lineColor\":\"#d95319\",\"parentID\":5326,\"plots\":[],\"port\":9,\"sid\":[\"\"],\"signalID\":5823,\"signalName\":\"packed_tw\"},\"type\":\"RecordBlkView.Signal\",\"uuid\":\"ab7e27e8-5321-4674-ba25-1205592251f9\"},{\"content\":{\"blockPath\":[\"SwarmSystem/Record\"],\"channel\":[9,3,2],\"dimensions\":[9,9,3],\"domain\":\"SwarmSystem/Record\",\"lineColor\":\"#edb120\",\"parentID\":5326,\"plots\":[],\"port\":9,\"sid\":[\"\"],\"signalID\":5824,\"signalName\":\"packed_tw\"},\"type\":\"RecordBlkView.Signal\",\"uuid\":\"d9834565-c616-4685-982e-2acf66321c2f\"},{\"content\":{\"blockPath\":[\"SwarmSystem/Record\"],\"channel\":[1,4,2],\"dimensions\":[9,9,3],\"domain\":\"SwarmSystem/Record\",\"lineColor\":\"#7e2f8e\",\"parentID\":5326,\"plots\":[],\"port\":9,\"sid\":[\"\"],\"signalID\":5825,\"signalName\":\"packed_tw\"},\"type\":\"RecordBlkView.Signal\",\"uuid\":\"73a8f051-ac54-418b-be34-57c1bea9c926\"},{\"content\":{\"blockPath\":[\"SwarmSystem/Record\"],\"channel\":[2,4,2],\"dimensions\":[9,9,3],\"domain\":\"SwarmSystem/Record\",\"lineColor\":\"#77ac30\",\"parentID\":5326,\"plots\":[],\"port\":9,\"sid\":[\"\"],\"signalID\":5826,\"signalName\":\"packed_tw\"},\"type\":\"RecordBlkView.Signal\",\"uuid\":\"ec901a96-64ba-450d-8db8-9e10e434bb41\"},{\"content\":{\"blockPath\":[\"SwarmSystem/Record\"],\"channel\":[3,4,2],\"dimensions\":[9,9,3],\"domain\":\"SwarmSystem/Record\",\"lineColor\":\"#4dbeee\",\"parentID\":5326,\"plots\":[],\"port\":9,\"sid\":[\"\"],\"signalID\":5827,\"signalName\":\"packed_tw\"},\"type\":\"RecordBlkView.Signal\",\"uuid\":\"534b9c5f-68be-4bd8-b4a6-75f5e7942e28\"},{\"content\":{\"blockPath\":[\"SwarmSystem/Record\"],\"channel\":[4,4,2],\"dimensions\":[9,9,3],\"domain\":\"SwarmSystem/Record\",\"lineColor\":\"#a2142f\",\"parentID\":5326,\"plots\":[],\"port\":9,\"sid\":[\"\"],\"signalID\":5828,\"signalName\":\"packed_tw\"},\"type\":\"RecordBlkView.Signal\",\"uuid\":\"57cb10d4-3295-407a-b4d9-6c20fce866fa\"},{\"content\":{\"blockPath\":[\"SwarmSystem/Record\"],\"channel\":[5,4,2],\"dimensions\":[9,9,3],\"domain\":\"SwarmSystem/Record\",\"lineColor\":\"#139fff\",\"parentID\":5326,\"plots\":[],\"port\":9,\"sid\":[\"\"],\"signalID\":5829,\"signalName\":\"packed_tw\"},\"type\":\"RecordBlkView.Signal\",\"uuid\":\"f5f3c6c1-4e62-4e43-b99f-60b52f41186b\"},{\"content\":{\"blockPath\":[\"SwarmSystem/Record\"],\"channel\":[6,4,2],\"dimensions\":[9,9,3],\"domain\":\"SwarmSystem/Record\",\"lineColor\":\"#ff6929\",\"parentID\":5326,\"plots\":[],\"port\":9,\"sid\":[\"\"],\"signalID\":5830,\"signalName\":\"packed_tw\"},\"type\":\"RecordBlkView.Signal\",\"uuid\":\"dc35dde6-03e7-4e6f-96f1-92d578fc4cc8\"},{\"content\":{\"blockPath\":[\"SwarmSystem/Record\"],\"channel\":[7,4,2],\"dimensions\":[9,9,3],\"domain\":\"SwarmSystem/Record\",\"lineColor\":\"#b746ff\",\"parentID\":5326,\"plots\":[],\"port\":9,\"sid\":[\"\"],\"signalID\":5831,\"signalName\":\"packed_tw\"},\"type\":\"RecordBlkView.Signal\",\"uuid\":\"fb50e130-57ac-4c05-99f1-ad9b0756c040\"},{\"content\":{\"blockPath\":[\"SwarmSystem/Record\"],\"channel\":[8,4,2],\"dimensions\":[9,9,3],\"domain\":\"SwarmSystem/Record\",\"lineColor\":\"#64d413\",\"parentID\":5326,\"plots\":[],\"port\":9,\"sid\":[\"\"],\"signalID\":5832,\"signalName\":\"packed_tw\"},\"type\":\"RecordBlkView.Signal\",\"uuid\":\"dba0bcf1-9b0a-48a3-aae0-fa7dbe3bde5c\"},{\"content\":{\"blockPath\":[\"SwarmSystem/Record\"],\"channel\":[9,4,2],\"dimensions\":[9,9,3],\"domain\":\"SwarmSystem/Record\",\"lineColor\":\"#ff13a6\",\"parentID\":5326,\"plots\":[],\"port\":9,\"sid\":[\"\"],\"signalID\":5833,\"signalName\":\"packed_tw\"},\"type\":\"RecordBlkView.Signal\",\"uuid\":\"1cebf3f3-22dc-42d8-be53-d17a558b4ebc\"},{\"content\":{\"blockPath\":[\"SwarmSystem/Record\"],\"channel\":[1,5,2],\"dimensions\":[9,9,3],\"domain\":\"SwarmSystem/Record\",\"lineColor\":\"#fe330a\",\"parentID\":5326,\"plots\":[],\"port\":9,\"sid\":[\"\"],\"signalID\":5834,\"signalName\":\"packed_tw\"},\"type\":\"RecordBlkView.Signal\",\"uuid\":\"4fa55bca-6c09-4e46-a298-f94e0ea4cde9\"},{\"content\":{\"blockPath\":[\"SwarmSystem/Record\"],\"channel\":[2,5,2],\"dimensions\":[9,9,3],\"domain\":\"SwarmSystem/Record\",\"lineColor\":\"#22b573\",\"parentID\":5326,\"plots\":[],\"port\":9,\"sid\":[\"\"],\"signalID\":5835,\"signalName\":\"packed_tw\"},\"type\":\"RecordBlkView.Signal\",\"uuid\":\"d9747375-d0b0-44d0-95bb-be2acc7336b4\"},{\"content\":{\"blockPath\":[\"SwarmSystem/Record\"],\"channel\":[3,5,2],\"dimensions\":[9,9,3],\"domain\":\"SwarmSystem/Record\",\"lineColor\":\"#0072bd\",\"parentID\":5326,\"plots\":[],\"port\":9,\"sid\":[\"\"],\"signalID\":5836,\"signalName\":\"packed_tw\"},\"type\":\"RecordBlkView.Signal\",\"uuid\":\"8fc234f2-8d4e-4730-aa50-051c53edd537\"},{\"content\":{\"blockPath\":[\"SwarmSystem/Record\"],\"channel\":[4,5,2],\"dimensions\":[9,9,3],\"domain\":\"SwarmSystem/Record\",\"lineColor\":\"#d95319\",\"parentID\":5326,\"plots\":[],\"port\":9,\"sid\":[\"\"],\"signalID\":5837,\"signalName\":\"packed_tw\"},\"type\":\"RecordBlkView.Signal\",\"uuid\":\"a560e1ad-7774-4d9f-84bb-5f05b7e7085f\"},{\"content\":{\"blockPath\":[\"SwarmSystem/Record\"],\"channel\":[5,5,2],\"dimensions\":[9,9,3],\"domain\":\"SwarmSystem/Record\",\"lineColor\":\"#edb120\",\"parentID\":5326,\"plots\":[],\"port\":9,\"sid\":[\"\"],\"signalID\":5838,\"signalName\":\"packed_tw\"},\"type\":\"RecordBlkView.Signal\",\"uuid\":\"fd6ffdc4-27b6-4286-a4fe-fc74007b7de1\"},{\"content\":{\"blockPath\":[\"SwarmSystem/Record\"],\"channel\":[6,5,2],\"dimensions\":[9,9,3],\"domain\":\"SwarmSystem/Record\",\"lineColor\":\"#7e2f8e\",\"parentID\":5326,\"plots\":[],\"port\":9,\"sid\":[\"\"],\"signalID\":5839,\"signalName\":\"packed_tw\"},\"type\":\"RecordBlkView.Signal\",\"uuid\":\"30fe91e8-e058-4076-8567-0aa02a5d7a8b\"},{\"content\":{\"blockPath\":[\"SwarmSystem/Record\"],\"channel\":[7,5,2],\"dimensions\":[9,9,3],\"domain\":\"SwarmSystem/Record\",\"lineColor\":\"#77ac30\",\"parentID\":5326,\"plots\":[],\"port\":9,\"sid\":[\"\"],\"signalID\":5840,\"signalName\":\"packed_tw\"},\"type\":\"RecordBlkView.Signal\",\"uuid\":\"4d8de427-c42c-47e2-9661-72de3c01d0ec\"},{\"content\":{\"blockPath\":[\"SwarmSystem/Record\"],\"channel\":[8,5,2],\"dimensions\":[9,9,3],\"domain\":\"SwarmSystem/Record\",\"lineColor\":\"#4dbeee\",\"parentID\":5326,\"plots\":[],\"port\":9,\"sid\":[\"\"],\"signalID\":5841,\"signalName\":\"packed_tw\"},\"type\":\"RecordBlkView.Signal\",\"uuid\":\"74cb2627-61cd-403d-a7f2-2a0ab0ef8735\"},{\"content\":{\"blockPath\":[\"SwarmSystem/Record\"],\"channel\":[9,5,2],\"dimensions\":[9,9,3],\"domain\":\"SwarmSystem/Record\",\"lineColor\":\"#a2142f\",\"parentID\":5326,\"plots\":[],\"port\":9,\"sid\":[\"\"],\"signalID\":5842,\"signalName\":\"packed_tw\"},\"type\":\"RecordBlkView.Signal\",\"uuid\":\"afaaa2ce-30f7-42df-9fa7-b477d412027f\"},{\"content\":{\"blockPath\":[\"SwarmSystem/Record\"],\"channel\":[1,6,2],\"dimensions\":[9,9,3],\"domain\":\"SwarmSystem/Record\",\"lineColor\":\"#139fff\",\"parentID\":5326,\"plots\":[],\"port\":9,\"sid\":[\"\"],\"signalID\":5843,\"signalName\":\"packed_tw\"},\"type\":\"RecordBlkView.Signal\",\"uuid\":\"2b9b8baf-bf8c-43d3-8545-d5dd11e917b6\"},{\"content\":{\"blockPath\":[\"SwarmSystem/Record\"],\"channel\":[2,6,2],\"dimensions\":[9,9,3],\"domain\":\"SwarmSystem/Record\",\"lineColor\":\"#ff6929\",\"parentID\":5326,\"plots\":[],\"port\":9,\"sid\":[\"\"],\"signalID\":5844,\"signalName\":\"packed_tw\"},\"type\":\"RecordBlkView.Signal\",\"uuid\":\"27da3e74-6207-4525-b469-5e6bde21a3cc\"},{\"content\":{\"blockPath\":[\"SwarmSystem/Record\"],\"channel\":[3,6,2],\"dimensions\":[9,9,3],\"domain\":\"SwarmSystem/Record\",\"lineColor\":\"#b746ff\",\"parentID\":5326,\"plots\":[],\"port\":9,\"sid\":[\"\"],\"signalID\":5845,\"signalName\":\"packed_tw\"},\"type\":\"RecordBlkView.Signal\",\"uuid\":\"ec549dc2-6e7b-4aa4-8717-32341151da85\"},{\"content\":{\"blockPath\":[\"SwarmSystem/Record\"],\"channel\":[4,6,2],\"dimensions\":[9,9,3],\"domain\":\"SwarmSystem/Record\",\"lineColor\":\"#64d413\",\"parentID\":5326,\"plots\":[],\"port\":9,\"sid\":[\"\"],\"signalID\":5846,\"signalName\":\"packed_tw\"},\"type\":\"RecordBlkView.Signal\",\"uuid\":\"3810786b-6fc5-447c-90fa-4501f974c104\"},{\"content\":{\"blockPath\":[\"SwarmSystem/Record\"],\"channel\":[5,6,2],\"dimensions\":[9,9,3],\"domain\":\"SwarmSystem/Record\",\"lineColor\":\"#ff13a6\",\"parentID\":5326,\"plots\":[],\"port\":9,\"sid\":[\"\"],\"signalID\":5847,\"signalName\":\"packed_tw\"},\"type\":\"RecordBlkView.Signal\",\"uuid\":\"350f9213-3236-42e0-9a84-c2d156ad98e5\"},{\"content\":{\"blockPath\":[\"SwarmSystem/Record\"],\"channel\":[6,6,2],\"dimensions\":[9,9,3],\"domain\":\"SwarmSystem/Record\",\"lineColor\":\"#fe330a\",\"parentID\":5326,\"plots\":[],\"port\":9,\"sid\":[\"\"],\"signalID\":5848,\"signalName\":\"packed_tw\"},\"type\":\"RecordBlkView.Signal\",\"uuid\":\"bf53ad8c-e4c8-4f8c-afce-f7cdaa2ca3d8\"},{\"content\":{\"blockPath\":[\"SwarmSystem/Record\"],\"channel\":[7,6,2],\"dimensions\":[9,9,3],\"domain\":\"SwarmSystem/Record\",\"lineColor\":\"#22b573\",\"parentID\":5326,\"plots\":[],\"port\":9,\"sid\":[\"\"],\"signalID\":5849,\"signalName\":\"packed_tw\"},\"type\":\"RecordBlkView.Signal\",\"uuid\":\"23223d4b-caaa-4fa7-ac98-d2259d2a24f9\"},{\"content\":{\"blockPath\":[\"SwarmSystem/Record\"],\"channel\":[8,6,2],\"dimensions\":[9,9,3],\"domain\":\"SwarmSystem/Record\",\"lineColor\":\"#0072bd\",\"parentID\":5326,\"plots\":[],\"port\":9,\"sid\":[\"\"],\"signalID\":5850,\"signalName\":\"packed_tw\"},\"type\":\"RecordBlkView.Signal\",\"uuid\":\"63030a99-4c11-4f54-b3d2-20de3edc01ae\"},{\"content\":{\"blockPath\":[\"SwarmSystem/Record\"],\"channel\":[9,6,2],\"dimensions\":[9,9,3],\"domain\":\"SwarmSystem/Record\",\"lineColor\":\"#d95319\",\"parentID\":5326,\"plots\":[],\"port\":9,\"sid\":[\"\"],\"signalID\":5851,\"signalName\":\"packed_tw\"},\"type\":\"RecordBlkView.Signal\",\"uuid\":\"daf11414-de17-40fd-b16f-9cef8180c3ce\"},{\"content\":{\"blockPath\":[\"SwarmSystem/Record\"],\"channel\":[1,7,2],\"dimensions\":[9,9,3],\"domain\":\"SwarmSystem/Record\",\"lineColor\":\"#edb120\",\"parentID\":5326,\"plots\":[],\"port\":9,\"sid\":[\"\"],\"signalID\":5852,\"signalName\":\"packed_tw\"},\"type\":\"RecordBlkView.Signal\",\"uuid\":\"5c216cbf-84a0-49ab-8b88-0e83cf29bb5b\"},{\"content\":{\"blockPath\":[\"SwarmSystem/Record\"],\"channel\":[2,7,2],\"dimensions\":[9,9,3],\"domain\":\"SwarmSystem/Record\",\"lineColor\":\"#7e2f8e\",\"parentID\":5326,\"plots\":[],\"port\":9,\"sid\":[\"\"],\"signalID\":5853,\"signalName\":\"packed_tw\"},\"type\":\"RecordBlkView.Signal\",\"uuid\":\"9a15c3a6-5876-4fb9-b452-713c30ffc3db\"},{\"content\":{\"blockPath\":[\"SwarmSystem/Record\"],\"channel\":[3,7,2],\"dimensions\":[9,9,3],\"domain\":\"SwarmSystem/Record\",\"lineColor\":\"#77ac30\",\"parentID\":5326,\"plots\":[],\"port\":9,\"sid\":[\"\"],\"signalID\":5854,\"signalName\":\"packed_tw\"},\"type\":\"RecordBlkView.Signal\",\"uuid\":\"77b04b48-d4fc-4539-b1bc-4a2498796ef9\"},{\"content\":{\"blockPath\":[\"SwarmSystem/Record\"],\"channel\":[4,7,2],\"dimensions\":[9,9,3],\"domain\":\"SwarmSystem/Record\",\"lineColor\":\"#4dbeee\",\"parentID\":5326,\"plots\":[],\"port\":9,\"sid\":[\"\"],\"signalID\":5855,\"signalName\":\"packed_tw\"},\"type\":\"RecordBlkView.Signal\",\"uuid\":\"54865afb-8fd3-4e9d-9a73-db6853d69f30\"},{\"content\":{\"blockPath\":[\"SwarmSystem/Record\"],\"channel\":[5,7,2],\"dimensions\":[9,9,3],\"domain\":\"SwarmSystem/Record\",\"lineColor\":\"#a2142f\",\"parentID\":5326,\"plots\":[],\"port\":9,\"sid\":[\"\"],\"signalID\":5856,\"signalName\":\"packed_tw\"},\"type\":\"RecordBlkView.Signal\",\"uuid\":\"5a37905a-7dc5-4129-9ddc-427332dceb3c\"},{\"content\":{\"blockPath\":[\"SwarmSystem/Record\"],\"channel\":[6,7,2],\"dimensions\":[9,9,3],\"domain\":\"SwarmSystem/Record\",\"lineColor\":\"#139fff\",\"parentID\":5326,\"plots\":[],\"port\":9,\"sid\":[\"\"],\"signalID\":5857,\"signalName\":\"packed_tw\"},\"type\":\"RecordBlkView.Signal\",\"uuid\":\"55e02785-f3c9-4f30-9e70-055683b503c6\"},{\"content\":{\"blockPath\":[\"SwarmSystem/Record\"],\"channel\":[7,7,2],\"dimensions\":[9,9,3],\"domain\":\"SwarmSystem/Record\",\"lineColor\":\"#ff6929\",\"parentID\":5326,\"plots\":[],\"port\":9,\"sid\":[\"\"],\"signalID\":5858,\"signalName\":\"packed_tw\"},\"type\":\"RecordBlkView.Signal\",\"uuid\":\"c4621d45-9f49-4b59-9860-d3cec35e13dc\"},{\"content\":{\"blockPath\":[\"SwarmSystem/Record\"],\"channel\":[8,7,2],\"dimensions\":[9,9,3],\"domain\":\"SwarmSystem/Record\",\"lineColor\":\"#b746ff\",\"parentID\":5326,\"plots\":[],\"port\":9,\"sid\":[\"\"],\"signalID\":5859,\"signalName\":\"packed_tw\"},\"type\":\"RecordBlkView.Signal\",\"uuid\":\"66bc8bcf-69e4-4a0c-83c3-778fe672c141\"},{\"content\":{\"blockPath\":[\"SwarmSystem/Record\"],\"channel\":[9,7,2],\"dimensions\":[9,9,3],\"domain\":\"SwarmSystem/Record\",\"lineColor\":\"#64d413\",\"parentID\":5326,\"plots\":[],\"port\":9,\"sid\":[\"\"],\"signalID\":5860,\"signalName\":\"packed_tw\"},\"type\":\"RecordBlkView.Signal\",\"uuid\":\"befc1550-8494-476a-9ad5-71573721cd34\"},{\"content\":{\"blockPath\":[\"SwarmSystem/Record\"],\"channel\":[1,8,2],\"dimensions\":[9,9,3],\"domain\":\"SwarmSystem/Record\",\"lineColor\":\"#ff13a6\",\"parentID\":5326,\"plots\":[],\"port\":9,\"sid\":[\"\"],\"signalID\":5861,\"signalName\":\"packed_tw\"},\"type\":\"RecordBlkView.Signal\",\"uuid\":\"89e7da80-7382-4823-930c-9425c76bbdbe\"},{\"content\":{\"blockPath\":[\"SwarmSystem/Record\"],\"channel\":[2,8,2],\"dimensions\":[9,9,3],\"domain\":\"SwarmSystem/Record\",\"lineColor\":\"#fe330a\",\"parentID\":5326,\"plots\":[],\"port\":9,\"sid\":[\"\"],\"signalID\":5862,\"signalName\":\"packed_tw\"},\"type\":\"RecordBlkView.Signal\",\"uuid\":\"78be11b5-4573-4106-bc42-830ca92602e3\"},{\"content\":{\"blockPath\":[\"SwarmSystem/Record\"],\"channel\":[3,8,2],\"dimensions\":[9,9,3],\"domain\":\"SwarmSystem/Record\",\"lineColor\":\"#22b573\",\"parentID\":5326,\"plots\":[],\"port\":9,\"sid\":[\"\"],\"signalID\":5863,\"signalName\":\"packed_tw\"},\"type\":\"RecordBlkView.Signal\",\"uuid\":\"985b922b-c6da-4ed8-9e7f-c8666a892499\"},{\"content\":{\"blockPath\":[\"SwarmSystem/Record\"],\"channel\":[4,8,2],\"dimensions\":[9,9,3],\"domain\":\"SwarmSystem/Record\",\"lineColor\":\"#0072bd\",\"parentID\":5326,\"plots\":[],\"port\":9,\"sid\":[\"\"],\"signalID\":5864,\"signalName\":\"packed_tw\"},\"type\":\"RecordBlkView.Signal\",\"uuid\":\"8318e3b6-aa64-493b-ba40-0f10a9dccc69\"},{\"content\":{\"blockPath\":[\"SwarmSystem/Record\"],\"channel\":[5,8,2],\"dimensions\":[9,9,3],\"domain\":\"SwarmSystem/Record\",\"lineColor\":\"#d95319\",\"parentID\":5326,\"plots\":[],\"port\":9,\"sid\":[\"\"],\"signalID\":5865,\"signalName\":\"packed_tw\"},\"type\":\"RecordBlkView.Signal\",\"uuid\":\"71f5a8dd-6b9b-4030-a3da-d55e24c9bd9d\"},{\"content\":{\"blockPath\":[\"SwarmSystem/Record\"],\"channel\":[6,8,2],\"dimensions\":[9,9,3],\"domain\":\"SwarmSystem/Record\",\"lineColor\":\"#edb120\",\"parentID\":5326,\"plots\":[],\"port\":9,\"sid\":[\"\"],\"signalID\":5866,\"signalName\":\"packed_tw\"},\"type\":\"RecordBlkView.Signal\",\"uuid\":\"dc2b2bbf-f1cc-4a75-ba9e-73d6ae689d06\"},{\"content\":{\"blockPath\":[\"SwarmSystem/Record\"],\"channel\":[7,8,2],\"dimensions\":[9,9,3],\"domain\":\"SwarmSystem/Record\",\"lineColor\":\"#7e2f8e\",\"parentID\":5326,\"plots\":[],\"port\":9,\"sid\":[\"\"],\"signalID\":5867,\"signalName\":\"packed_tw\"},\"type\":\"RecordBlkView.Signal\",\"uuid\":\"83de003e-5e66-48f7-a58e-dd4f21d6dee3\"},{\"content\":{\"blockPath\":[\"SwarmSystem/Record\"],\"channel\":[8,8,2],\"dimensions\":[9,9,3],\"domain\":\"SwarmSystem/Record\",\"lineColor\":\"#77ac30\",\"parentID\":5326,\"plots\":[],\"port\":9,\"sid\":[\"\"],\"signalID\":5868,\"signalName\":\"packed_tw\"},\"type\":\"RecordBlkView.Signal\",\"uuid\":\"6a4ae856-4224-42f6-ab6c-cf77b60fe43f\"},{\"content\":{\"blockPath\":[\"SwarmSystem/Record\"],\"channel\":[9,8,2],\"dimensions\":[9,9,3],\"domain\":\"SwarmSystem/Record\",\"lineColor\":\"#4dbeee\",\"parentID\":5326,\"plots\":[],\"port\":9,\"sid\":[\"\"],\"signalID\":5869,\"signalName\":\"packed_tw\"},\"type\":\"RecordBlkView.Signal\",\"uuid\":\"70287095-a51d-465c-96bd-95abfff14d85\"},{\"content\":{\"blockPath\":[\"SwarmSystem/Record\"],\"channel\":[1,9,2],\"dimensions\":[9,9,3],\"domain\":\"SwarmSystem/Record\",\"lineColor\":\"#a2142f\",\"parentID\":5326,\"plots\":[],\"port\":9,\"sid\":[\"\"],\"signalID\":5870,\"signalName\":\"packed_tw\"},\"type\":\"RecordBlkView.Signal\",\"uuid\":\"f7d32c7b-66e7-4403-85cf-fdc09158aca6\"},{\"content\":{\"blockPath\":[\"SwarmSystem/Record\"],\"channel\":[2,9,2],\"dimensions\":[9,9,3],\"domain\":\"SwarmSystem/Record\",\"lineColor\":\"#139fff\",\"parentID\":5326,\"plots\":[],\"port\":9,\"sid\":[\"\"],\"signalID\":5871,\"signalName\":\"packed_tw\"},\"type\":\"RecordBlkView.Signal\",\"uuid\":\"d0231013-ae14-437c-a7bf-7c256498311a\"},{\"content\":{\"blockPath\":[\"SwarmSystem/Record\"],\"channel\":[3,9,2],\"dimensions\":[9,9,3],\"domain\":\"SwarmSystem/Record\",\"lineColor\":\"#ff6929\",\"parentID\":5326,\"plots\":[],\"port\":9,\"sid\":[\"\"],\"signalID\":5872,\"signalName\":\"packed_tw\"},\"type\":\"RecordBlkView.Signal\",\"uuid\":\"61b38bb1-158b-4496-b252-314e654ee7b1\"},{\"content\":{\"blockPath\":[\"SwarmSystem/Record\"],\"channel\":[4,9,2],\"dimensions\":[9,9,3],\"domain\":\"SwarmSystem/Record\",\"lineColor\":\"#b746ff\",\"parentID\":5326,\"plots\":[],\"port\":9,\"sid\":[\"\"],\"signalID\":5873,\"signalName\":\"packed_tw\"},\"type\":\"RecordBlkView.Signal\",\"uuid\":\"3bcbd5d8-db97-44f9-9b50-d99b0e2a4307\"},{\"content\":{\"blockPath\":[\"SwarmSystem/Record\"],\"channel\":[5,9,2],\"dimensions\":[9,9,3],\"domain\":\"SwarmSystem/Record\",\"lineColor\":\"#64d413\",\"parentID\":5326,\"plots\":[],\"port\":9,\"sid\":[\"\"],\"signalID\":5874,\"signalName\":\"packed_tw\"},\"type\":\"RecordBlkView.Signal\",\"uuid\":\"f34a9d59-9d42-4e7b-b124-8c15edd15156\"},{\"content\":{\"blockPath\":[\"SwarmSystem/Record\"],\"channel\":[6,9,2],\"dimensions\":[9,9,3],\"domain\":\"SwarmSystem/Record\",\"lineColor\":\"#ff13a6\",\"parentID\":5326,\"plots\":[],\"port\":9,\"sid\":[\"\"],\"signalID\":5875,\"signalName\":\"packed_tw\"},\"type\":\"RecordBlkView.Signal\",\"uuid\":\"56aa242d-f87c-4f9d-9851-5391d0d6e15a\"},{\"content\":{\"blockPath\":[\"SwarmSystem/Record\"],\"channel\":[7,9,2],\"dimensions\":[9,9,3],\"domain\":\"SwarmSystem/Record\",\"lineColor\":\"#fe330a\",\"parentID\":5326,\"plots\":[],\"port\":9,\"sid\":[\"\"],\"signalID\":5876,\"signalName\":\"packed_tw\"},\"type\":\"RecordBlkView.Signal\",\"uuid\":\"ec21145f-b956-438f-9821-702e38fb14ca\"},{\"content\":{\"blockPath\":[\"SwarmSystem/Record\"],\"channel\":[8,9,2],\"dimensions\":[9,9,3],\"domain\":\"SwarmSystem/Record\",\"lineColor\":\"#22b573\",\"parentID\":5326,\"plots\":[],\"port\":9,\"sid\":[\"\"],\"signalID\":5877,\"signalName\":\"packed_tw\"},\"type\":\"RecordBlkView.Signal\",\"uuid\":\"cf375325-5cd0-4412-89e7-5c8eb8bee119\"},{\"content\":{\"blockPath\":[\"SwarmSystem/Record\"],\"channel\":[9,9,2],\"dimensions\":[9,9,3],\"domain\":\"SwarmSystem/Record\",\"lineColor\":\"#0072bd\",\"parentID\":5326,\"plots\":[],\"port\":9,\"sid\":[\"\"],\"signalID\":5878,\"signalName\":\"packed_tw\"},\"type\":\"RecordBlkView.Signal\",\"uuid\":\"b95e2f74-4f18-4661-b937-92eb628141f5\"},{\"content\":{\"blockPath\":[\"SwarmSystem/Record\"],\"channel\":[1,1,3],\"dimensions\":[9,9,3],\"domain\":\"SwarmSystem/Record\",\"lineColor\":\"#d95319\",\"parentID\":5326,\"plots\":[],\"port\":9,\"sid\":[\"\"],\"signalID\":5879,\"signalName\":\"packed_tw\"},\"type\":\"RecordBlkView.Signal\",\"uuid\":\"c182bea3-6275-4704-803f-f71501ba775b\"},{\"content\":{\"blockPath\":[\"SwarmSystem/Record\"],\"channel\":[2,1,3],\"dimensions\":[9,9,3],\"domain\":\"SwarmSystem/Record\",\"lineColor\":\"#edb120\",\"parentID\":5326,\"plots\":[],\"port\":9,\"sid\":[\"\"],\"signalID\":5880,\"signalName\":\"packed_tw\"},\"type\":\"RecordBlkView.Signal\",\"uuid\":\"d4aa9dd3-bb8d-4183-99c3-1fd40f695c42\"},{\"content\":{\"blockPath\":[\"SwarmSystem/Record\"],\"channel\":[3,1,3],\"dimensions\":[9,9,3],\"domain\":\"SwarmSystem/Record\",\"lineColor\":\"#7e2f8e\",\"parentID\":5326,\"plots\":[],\"port\":9,\"sid\":[\"\"],\"signalID\":5881,\"signalName\":\"packed_tw\"},\"type\":\"RecordBlkView.Signal\",\"uuid\":\"506cd9d7-ea3f-4f14-9b9d-30b91182cdf1\"},{\"content\":{\"blockPath\":[\"SwarmSystem/Record\"],\"channel\":[4,1,3],\"dimensions\":[9,9,3],\"domain\":\"SwarmSystem/Record\",\"lineColor\":\"#77ac30\",\"parentID\":5326,\"plots\":[],\"port\":9,\"sid\":[\"\"],\"signalID\":5882,\"signalName\":\"packed_tw\"},\"type\":\"RecordBlkView.Signal\",\"uuid\":\"1ee1a467-c6bb-42e5-a7b9-4c614750e104\"},{\"content\":{\"blockPath\":[\"SwarmSystem/Record\"],\"channel\":[5,1,3],\"dimensions\":[9,9,3],\"domain\":\"SwarmSystem/Record\",\"lineColor\":\"#4dbeee\",\"parentID\":5326,\"plots\":[],\"port\":9,\"sid\":[\"\"],\"signalID\":5883,\"signalName\":\"packed_tw\"},\"type\":\"RecordBlkView.Signal\",\"uuid\":\"c430b5c4-2783-46c7-8f95-574efcf2cb6d\"},{\"content\":{\"blockPath\":[\"SwarmSystem/Record\"],\"channel\":[6,1,3],\"dimensions\":[9,9,3],\"domain\":\"SwarmSystem/Record\",\"lineColor\":\"#a2142f\",\"parentID\":5326,\"plots\":[],\"port\":9,\"sid\":[\"\"],\"signalID\":5884,\"signalName\":\"packed_tw\"},\"type\":\"RecordBlkView.Signal\",\"uuid\":\"1c4c8aab-15a8-4fac-8842-da3328c0cb71\"},{\"content\":{\"blockPath\":[\"SwarmSystem/Record\"],\"channel\":[7,1,3],\"dimensions\":[9,9,3],\"domain\":\"SwarmSystem/Record\",\"lineColor\":\"#139fff\",\"parentID\":5326,\"plots\":[],\"port\":9,\"sid\":[\"\"],\"signalID\":5885,\"signalName\":\"packed_tw\"},\"type\":\"RecordBlkView.Signal\",\"uuid\":\"636fe1c5-7c69-4767-9305-6ae51aab512f\"},{\"content\":{\"blockPath\":[\"SwarmSystem/Record\"],\"channel\":[8,1,3],\"dimensions\":[9,9,3],\"domain\":\"SwarmSystem/Record\",\"lineColor\":\"#ff6929\",\"parentID\":5326,\"plots\":[],\"port\":9,\"sid\":[\"\"],\"signalID\":5886,\"signalName\":\"packed_tw\"},\"type\":\"RecordBlkView.Signal\",\"uuid\":\"137d1df2-37c8-48fa-afc7-332910a2d68d\"},{\"content\":{\"blockPath\":[\"SwarmSystem/Record\"],\"channel\":[9,1,3],\"dimensions\":[9,9,3],\"domain\":\"SwarmSystem/Record\",\"lineColor\":\"#b746ff\",\"parentID\":5326,\"plots\":[],\"port\":9,\"sid\":[\"\"],\"signalID\":5887,\"signalName\":\"packed_tw\"},\"type\":\"RecordBlkView.Signal\",\"uuid\":\"bf074b16-294b-420a-b9e3-3be8396439b3\"},{\"content\":{\"blockPath\":[\"SwarmSystem/Record\"],\"channel\":[1,2,3],\"dimensions\":[9,9,3],\"domain\":\"SwarmSystem/Record\",\"lineColor\":\"#64d413\",\"parentID\":5326,\"plots\":[],\"port\":9,\"sid\":[\"\"],\"signalID\":5888,\"signalName\":\"packed_tw\"},\"type\":\"RecordBlkView.Signal\",\"uuid\":\"97488361-5f33-4832-b8d5-b64d25f32c9f\"},{\"content\":{\"blockPath\":[\"SwarmSystem/Record\"],\"channel\":[2,2,3],\"dimensions\":[9,9,3],\"domain\":\"SwarmSystem/Record\",\"lineColor\":\"#ff13a6\",\"parentID\":5326,\"plots\":[],\"port\":9,\"sid\":[\"\"],\"signalID\":5889,\"signalName\":\"packed_tw\"},\"type\":\"RecordBlkView.Signal\",\"uuid\":\"5ea6e07f-fe06-4071-81cc-80a62288da15\"},{\"content\":{\"blockPath\":[\"SwarmSystem/Record\"],\"channel\":[3,2,3],\"dimensions\":[9,9,3],\"domain\":\"SwarmSystem/Record\",\"lineColor\":\"#fe330a\",\"parentID\":5326,\"plots\":[],\"port\":9,\"sid\":[\"\"],\"signalID\":5890,\"signalName\":\"packed_tw\"},\"type\":\"RecordBlkView.Signal\",\"uuid\":\"4cefdf24-f504-4ff6-a03f-1a4de9a8b572\"},{\"content\":{\"blockPath\":[\"SwarmSystem/Record\"],\"channel\":[4,2,3],\"dimensions\":[9,9,3],\"domain\":\"SwarmSystem/Record\",\"lineColor\":\"#22b573\",\"parentID\":5326,\"plots\":[],\"port\":9,\"sid\":[\"\"],\"signalID\":5891,\"signalName\":\"packed_tw\"},\"type\":\"RecordBlkView.Signal\",\"uuid\":\"eafd0c49-3242-41c0-9b88-d483e5e7fe73\"},{\"content\":{\"blockPath\":[\"SwarmSystem/Record\"],\"channel\":[5,2,3],\"dimensions\":[9,9,3],\"domain\":\"SwarmSystem/Record\",\"lineColor\":\"#0072bd\",\"parentID\":5326,\"plots\":[],\"port\":9,\"sid\":[\"\"],\"signalID\":5892,\"signalName\":\"packed_tw\"},\"type\":\"RecordBlkView.Signal\",\"uuid\":\"33ae9641-f7a3-4236-b300-55aca3511789\"},{\"content\":{\"blockPath\":[\"SwarmSystem/Record\"],\"channel\":[6,2,3],\"dimensions\":[9,9,3],\"domain\":\"SwarmSystem/Record\",\"lineColor\":\"#d95319\",\"parentID\":5326,\"plots\":[],\"port\":9,\"sid\":[\"\"],\"signalID\":5893,\"signalName\":\"packed_tw\"},\"type\":\"RecordBlkView.Signal\",\"uuid\":\"2be64d80-aff3-4406-8a86-63938a0f6943\"},{\"content\":{\"blockPath\":[\"SwarmSystem/Record\"],\"channel\":[7,2,3],\"dimensions\":[9,9,3],\"domain\":\"SwarmSystem/Record\",\"lineColor\":\"#edb120\",\"parentID\":5326,\"plots\":[],\"port\":9,\"sid\":[\"\"],\"signalID\":5894,\"signalName\":\"packed_tw\"},\"type\":\"RecordBlkView.Signal\",\"uuid\":\"512f272c-484b-45b0-a649-e3125e1db2d2\"},{\"content\":{\"blockPath\":[\"SwarmSystem/Record\"],\"channel\":[8,2,3],\"dimensions\":[9,9,3],\"domain\":\"SwarmSystem/Record\",\"lineColor\":\"#7e2f8e\",\"parentID\":5326,\"plots\":[],\"port\":9,\"sid\":[\"\"],\"signalID\":5895,\"signalName\":\"packed_tw\"},\"type\":\"RecordBlkView.Signal\",\"uuid\":\"ba9768ab-b306-4f09-9e2c-b8b91d93b48d\"},{\"content\":{\"blockPath\":[\"SwarmSystem/Record\"],\"channel\":[9,2,3],\"dimensions\":[9,9,3],\"domain\":\"SwarmSystem/Record\",\"lineColor\":\"#77ac30\",\"parentID\":5326,\"plots\":[],\"port\":9,\"sid\":[\"\"],\"signalID\":5896,\"signalName\":\"packed_tw\"},\"type\":\"RecordBlkView.Signal\",\"uuid\":\"700578dc-1616-4acc-9b51-3067b03f233c\"},{\"content\":{\"blockPath\":[\"SwarmSystem/Record\"],\"channel\":[1,3,3],\"dimensions\":[9,9,3],\"domain\":\"SwarmSystem/Record\",\"lineColor\":\"#4dbeee\",\"parentID\":5326,\"plots\":[],\"port\":9,\"sid\":[\"\"],\"signalID\":5897,\"signalName\":\"packed_tw\"},\"type\":\"RecordBlkView.Signal\",\"uuid\":\"e44b8eb4-3187-4b25-84e6-baeeec1e27e2\"},{\"content\":{\"blockPath\":[\"SwarmSystem/Record\"],\"channel\":[2,3,3],\"dimensions\":[9,9,3],\"domain\":\"SwarmSystem/Record\",\"lineColor\":\"#a2142f\",\"parentID\":5326,\"plots\":[],\"port\":9,\"sid\":[\"\"],\"signalID\":5898,\"signalName\":\"packed_tw\"},\"type\":\"RecordBlkView.Signal\",\"uuid\":\"76720af5-7096-4b1e-b282-0e2fae0dc669\"},{\"content\":{\"blockPath\":[\"SwarmSystem/Record\"],\"channel\":[3,3,3],\"dimensions\":[9,9,3],\"domain\":\"SwarmSystem/Record\",\"lineColor\":\"#139fff\",\"parentID\":5326,\"plots\":[],\"port\":9,\"sid\":[\"\"],\"signalID\":5899,\"signalName\":\"packed_tw\"},\"type\":\"RecordBlkView.Signal\",\"uuid\":\"01380df4-5af0-407f-a963-c1856c7dc8e1\"},{\"content\":{\"blockPath\":[\"SwarmSystem/Record\"],\"channel\":[4,3,3],\"dimensions\":[9,9,3],\"domain\":\"SwarmSystem/Record\",\"lineColor\":\"#ff6929\",\"parentID\":5326,\"plots\":[],\"port\":9,\"sid\":[\"\"],\"signalID\":5900,\"signalName\":\"packed_tw\"},\"type\":\"RecordBlkView.Signal\",\"uuid\":\"58ed861f-a0e7-4d30-ac5d-b4db70b9ff04\"},{\"content\":{\"blockPath\":[\"SwarmSystem/Record\"],\"channel\":[5,3,3],\"dimensions\":[9,9,3],\"domain\":\"SwarmSystem/Record\",\"lineColor\":\"#b746ff\",\"parentID\":5326,\"plots\":[],\"port\":9,\"sid\":[\"\"],\"signalID\":5901,\"signalName\":\"packed_tw\"},\"type\":\"RecordBlkView.Signal\",\"uuid\":\"1b4f9c69-a014-4abc-bb13-21be5a13954f\"},{\"content\":{\"blockPath\":[\"SwarmSystem/Record\"],\"channel\":[6,3,3],\"dimensions\":[9,9,3],\"domain\":\"SwarmSystem/Record\",\"lineColor\":\"#64d413\",\"parentID\":5326,\"plots\":[],\"port\":9,\"sid\":[\"\"],\"signalID\":5902,\"signalName\":\"packed_tw\"},\"type\":\"RecordBlkView.Signal\",\"uuid\":\"6c56f590-c4c4-40ab-b1a7-ba4891fdd94d\"},{\"content\":{\"blockPath\":[\"SwarmSystem/Record\"],\"channel\":[7,3,3],\"dimensions\":[9,9,3],\"domain\":\"SwarmSystem/Record\",\"lineColor\":\"#ff13a6\",\"parentID\":5326,\"plots\":[],\"port\":9,\"sid\":[\"\"],\"signalID\":5903,\"signalName\":\"packed_tw\"},\"type\":\"RecordBlkView.Signal\",\"uuid\":\"9cff10c2-69ff-4ec0-8e2d-b2f0062826f6\"},{\"content\":{\"blockPath\":[\"SwarmSystem/Record\"],\"channel\":[8,3,3],\"dimensions\":[9,9,3],\"domain\":\"SwarmSystem/Record\",\"lineColor\":\"#fe330a\",\"parentID\":5326,\"plots\":[],\"port\":9,\"sid\":[\"\"],\"signalID\":5904,\"signalName\":\"packed_tw\"},\"type\":\"RecordBlkView.Signal\",\"uuid\":\"e70ed971-40b1-4941-95be-99d520d6c269\"},{\"content\":{\"blockPath\":[\"SwarmSystem/Record\"],\"channel\":[9,3,3],\"dimensions\":[9,9,3],\"domain\":\"SwarmSystem/Record\",\"lineColor\":\"#22b573\",\"parentID\":5326,\"plots\":[],\"port\":9,\"sid\":[\"\"],\"signalID\":5905,\"signalName\":\"packed_tw\"},\"type\":\"RecordBlkView.Signal\",\"uuid\":\"6f6fbef9-f00e-48b0-bcc3-679d076b6b18\"},{\"content\":{\"blockPath\":[\"SwarmSystem/Record\"],\"channel\":[1,4,3],\"dimensions\":[9,9,3],\"domain\":\"SwarmSystem/Record\",\"lineColor\":\"#0072bd\",\"parentID\":5326,\"plots\":[],\"port\":9,\"sid\":[\"\"],\"signalID\":5906,\"signalName\":\"packed_tw\"},\"type\":\"RecordBlkView.Signal\",\"uuid\":\"7d69bb9c-0c55-498b-9861-fa8db9e23777\"},{\"content\":{\"blockPath\":[\"SwarmSystem/Record\"],\"channel\":[2,4,3],\"dimensions\":[9,9,3],\"domain\":\"SwarmSystem/Record\",\"lineColor\":\"#d95319\",\"parentID\":5326,\"plots\":[],\"port\":9,\"sid\":[\"\"],\"signalID\":5907,\"signalName\":\"packed_tw\"},\"type\":\"RecordBlkView.Signal\",\"uuid\":\"e56aaf64-be07-4e05-8f73-3bd6c5f77849\"},{\"content\":{\"blockPath\":[\"SwarmSystem/Record\"],\"channel\":[3,4,3],\"dimensions\":[9,9,3],\"domain\":\"SwarmSystem/Record\",\"lineColor\":\"#edb120\",\"parentID\":5326,\"plots\":[],\"port\":9,\"sid\":[\"\"],\"signalID\":5908,\"signalName\":\"packed_tw\"},\"type\":\"RecordBlkView.Signal\",\"uuid\":\"351a5eed-6b2f-4214-8e6b-a53f92502307\"},{\"content\":{\"blockPath\":[\"SwarmSystem/Record\"],\"channel\":[4,4,3],\"dimensions\":[9,9,3],\"domain\":\"SwarmSystem/Record\",\"lineColor\":\"#7e2f8e\",\"parentID\":5326,\"plots\":[],\"port\":9,\"sid\":[\"\"],\"signalID\":5909,\"signalName\":\"packed_tw\"},\"type\":\"RecordBlkView.Signal\",\"uuid\":\"183d5031-f03a-45bc-9b0f-0433b774dc00\"},{\"content\":{\"blockPath\":[\"SwarmSystem/Record\"],\"channel\":[5,4,3],\"dimensions\":[9,9,3],\"domain\":\"SwarmSystem/Record\",\"lineColor\":\"#77ac30\",\"parentID\":5326,\"plots\":[],\"port\":9,\"sid\":[\"\"],\"signalID\":5910,\"signalName\":\"packed_tw\"},\"type\":\"RecordBlkView.Signal\",\"uuid\":\"5f8b5a27-2603-4bca-b1bd-4cca560ee4d0\"},{\"content\":{\"blockPath\":[\"SwarmSystem/Record\"],\"channel\":[6,4,3],\"dimensions\":[9,9,3],\"domain\":\"SwarmSystem/Record\",\"lineColor\":\"#4dbeee\",\"parentID\":5326,\"plots\":[],\"port\":9,\"sid\":[\"\"],\"signalID\":5911,\"signalName\":\"packed_tw\"},\"type\":\"RecordBlkView.Signal\",\"uuid\":\"dd8208a6-771b-451c-9b55-fe7db679cf13\"},{\"content\":{\"blockPath\":[\"SwarmSystem/Record\"],\"channel\":[7,4,3],\"dimensions\":[9,9,3],\"domain\":\"SwarmSystem/Record\",\"lineColor\":\"#a2142f\",\"parentID\":5326,\"plots\":[],\"port\":9,\"sid\":[\"\"],\"signalID\":5912,\"signalName\":\"packed_tw\"},\"type\":\"RecordBlkView.Signal\",\"uuid\":\"dbc0dddb-bc16-444a-9219-0c225fd827c1\"},{\"content\":{\"blockPath\":[\"SwarmSystem/Record\"],\"channel\":[8,4,3],\"dimensions\":[9,9,3],\"domain\":\"SwarmSystem/Record\",\"lineColor\":\"#139fff\",\"parentID\":5326,\"plots\":[],\"port\":9,\"sid\":[\"\"],\"signalID\":5913,\"signalName\":\"packed_tw\"},\"type\":\"RecordBlkView.Signal\",\"uuid\":\"78da423a-fde9-4196-aaca-8274dac83e9a\"},{\"content\":{\"blockPath\":[\"SwarmSystem/Record\"],\"channel\":[9,4,3],\"dimensions\":[9,9,3],\"domain\":\"SwarmSystem/Record\",\"lineColor\":\"#ff6929\",\"parentID\":5326,\"plots\":[],\"port\":9,\"sid\":[\"\"],\"signalID\":5914,\"signalName\":\"packed_tw\"},\"type\":\"RecordBlkView.Signal\",\"uuid\":\"41b0067a-a89d-468a-995f-7d1e5b1a87ae\"},{\"content\":{\"blockPath\":[\"SwarmSystem/Record\"],\"channel\":[1,5,3],\"dimensions\":[9,9,3],\"domain\":\"SwarmSystem/Record\",\"lineColor\":\"#b746ff\",\"parentID\":5326,\"plots\":[],\"port\":9,\"sid\":[\"\"],\"signalID\":5915,\"signalName\":\"packed_tw\"},\"type\":\"RecordBlkView.Signal\",\"uuid\":\"be55a03a-d421-4928-bd18-089a4a8f2e53\"},{\"content\":{\"blockPath\":[\"SwarmSystem/Record\"],\"channel\":[2,5,3],\"dimensions\":[9,9,3],\"domain\":\"SwarmSystem/Record\",\"lineColor\":\"#64d413\",\"parentID\":5326,\"plots\":[],\"port\":9,\"sid\":[\"\"],\"signalID\":5916,\"signalName\":\"packed_tw\"},\"type\":\"RecordBlkView.Signal\",\"uuid\":\"c60d26f1-f16a-44f9-af2b-66db6d941118\"},{\"content\":{\"blockPath\":[\"SwarmSystem/Record\"],\"channel\":[3,5,3],\"dimensions\":[9,9,3],\"domain\":\"SwarmSystem/Record\",\"lineColor\":\"#ff13a6\",\"parentID\":5326,\"plots\":[],\"port\":9,\"sid\":[\"\"],\"signalID\":5917,\"signalName\":\"packed_tw\"},\"type\":\"RecordBlkView.Signal\",\"uuid\":\"f2da83ea-680c-4af8-b710-2978024cd939\"},{\"content\":{\"blockPath\":[\"SwarmSystem/Record\"],\"channel\":[4,5,3],\"dimensions\":[9,9,3],\"domain\":\"SwarmSystem/Record\",\"lineColor\":\"#fe330a\",\"parentID\":5326,\"plots\":[],\"port\":9,\"sid\":[\"\"],\"signalID\":5918,\"signalName\":\"packed_tw\"},\"type\":\"RecordBlkView.Signal\",\"uuid\":\"f4c832ba-c87b-4e10-b5c6-872fc1aa3c61\"},{\"content\":{\"blockPath\":[\"SwarmSystem/Record\"],\"channel\":[5,5,3],\"dimensions\":[9,9,3],\"domain\":\"SwarmSystem/Record\",\"lineColor\":\"#22b573\",\"parentID\":5326,\"plots\":[],\"port\":9,\"sid\":[\"\"],\"signalID\":5919,\"signalName\":\"packed_tw\"},\"type\":\"RecordBlkView.Signal\",\"uuid\":\"574ee972-52bc-46f0-af8d-8f351fcfca81\"},{\"content\":{\"blockPath\":[\"SwarmSystem/Record\"],\"channel\":[6,5,3],\"dimensions\":[9,9,3],\"domain\":\"SwarmSystem/Record\",\"lineColor\":\"#0072bd\",\"parentID\":5326,\"plots\":[],\"port\":9,\"sid\":[\"\"],\"signalID\":5920,\"signalName\":\"packed_tw\"},\"type\":\"RecordBlkView.Signal\",\"uuid\":\"a11f86a1-0253-495a-90a0-d23c041eb3d6\"},{\"content\":{\"blockPath\":[\"SwarmSystem/Record\"],\"channel\":[7,5,3],\"dimensions\":[9,9,3],\"domain\":\"SwarmSystem/Record\",\"lineColor\":\"#d95319\",\"parentID\":5326,\"plots\":[],\"port\":9,\"sid\":[\"\"],\"signalID\":5921,\"signalName\":\"packed_tw\"},\"type\":\"RecordBlkView.Signal\",\"uuid\":\"360f3a55-ee29-447f-ae7e-8e100cca612a\"},{\"content\":{\"blockPath\":[\"SwarmSystem/Record\"],\"channel\":[8,5,3],\"dimensions\":[9,9,3],\"domain\":\"SwarmSystem/Record\",\"lineColor\":\"#edb120\",\"parentID\":5326,\"plots\":[],\"port\":9,\"sid\":[\"\"],\"signalID\":5922,\"signalName\":\"packed_tw\"},\"type\":\"RecordBlkView.Signal\",\"uuid\":\"e7469b9f-e18a-40e2-8050-cf56c30ae475\"},{\"content\":{\"blockPath\":[\"SwarmSystem/Record\"],\"channel\":[9,5,3],\"dimensions\":[9,9,3],\"domain\":\"SwarmSystem/Record\",\"lineColor\":\"#7e2f8e\",\"parentID\":5326,\"plots\":[],\"port\":9,\"sid\":[\"\"],\"signalID\":5923,\"signalName\":\"packed_tw\"},\"type\":\"RecordBlkView.Signal\",\"uuid\":\"35b98bc3-279a-4580-af0b-8c5a865d31e8\"},{\"content\":{\"blockPath\":[\"SwarmSystem/Record\"],\"channel\":[1,6,3],\"dimensions\":[9,9,3],\"domain\":\"SwarmSystem/Record\",\"lineColor\":\"#77ac30\",\"parentID\":5326,\"plots\":[],\"port\":9,\"sid\":[\"\"],\"signalID\":5924,\"signalName\":\"packed_tw\"},\"type\":\"RecordBlkView.Signal\",\"uuid\":\"389f53a5-1158-4e01-a8a4-9b3d8051147f\"},{\"content\":{\"blockPath\":[\"SwarmSystem/Record\"],\"channel\":[2,6,3],\"dimensions\":[9,9,3],\"domain\":\"SwarmSystem/Record\",\"lineColor\":\"#4dbeee\",\"parentID\":5326,\"plots\":[],\"port\":9,\"sid\":[\"\"],\"signalID\":5925,\"signalName\":\"packed_tw\"},\"type\":\"RecordBlkView.Signal\",\"uuid\":\"cde5e527-3710-44ee-821a-aca3f0615818\"},{\"content\":{\"blockPath\":[\"SwarmSystem/Record\"],\"channel\":[3,6,3],\"dimensions\":[9,9,3],\"domain\":\"SwarmSystem/Record\",\"lineColor\":\"#a2142f\",\"parentID\":5326,\"plots\":[],\"port\":9,\"sid\":[\"\"],\"signalID\":5926,\"signalName\":\"packed_tw\"},\"type\":\"RecordBlkView.Signal\",\"uuid\":\"2f55b377-3ec3-4844-b4e7-68acae7f9290\"},{\"content\":{\"blockPath\":[\"SwarmSystem/Record\"],\"channel\":[4,6,3],\"dimensions\":[9,9,3],\"domain\":\"SwarmSystem/Record\",\"lineColor\":\"#139fff\",\"parentID\":5326,\"plots\":[],\"port\":9,\"sid\":[\"\"],\"signalID\":5927,\"signalName\":\"packed_tw\"},\"type\":\"RecordBlkView.Signal\",\"uuid\":\"538824cb-4687-4a87-ac7c-8915739b928f\"},{\"content\":{\"blockPath\":[\"SwarmSystem/Record\"],\"channel\":[5,6,3],\"dimensions\":[9,9,3],\"domain\":\"SwarmSystem/Record\",\"lineColor\":\"#ff6929\",\"parentID\":5326,\"plots\":[],\"port\":9,\"sid\":[\"\"],\"signalID\":5928,\"signalName\":\"packed_tw\"},\"type\":\"RecordBlkView.Signal\",\"uuid\":\"04ae4cf6-f53c-4ea4-ae40-12de55d23b0a\"},{\"content\":{\"blockPath\":[\"SwarmSystem/Record\"],\"channel\":[6,6,3],\"dimensions\":[9,9,3],\"domain\":\"SwarmSystem/Record\",\"lineColor\":\"#b746ff\",\"parentID\":5326,\"plots\":[],\"port\":9,\"sid\":[\"\"],\"signalID\":5929,\"signalName\":\"packed_tw\"},\"type\":\"RecordBlkView.Signal\",\"uuid\":\"67ea196e-63a4-4315-9138-6d962679371a\"},{\"content\":{\"blockPath\":[\"SwarmSystem/Record\"],\"channel\":[7,6,3],\"dimensions\":[9,9,3],\"domain\":\"SwarmSystem/Record\",\"lineColor\":\"#64d413\",\"parentID\":5326,\"plots\":[],\"port\":9,\"sid\":[\"\"],\"signalID\":5930,\"signalName\":\"packed_tw\"},\"type\":\"RecordBlkView.Signal\",\"uuid\":\"20b131db-262e-4f4f-a602-fed390a44f0f\"},{\"content\":{\"blockPath\":[\"SwarmSystem/Record\"],\"channel\":[8,6,3],\"dimensions\":[9,9,3],\"domain\":\"SwarmSystem/Record\",\"lineColor\":\"#ff13a6\",\"parentID\":5326,\"plots\":[],\"port\":9,\"sid\":[\"\"],\"signalID\":5931,\"signalName\":\"packed_tw\"},\"type\":\"RecordBlkView.Signal\",\"uuid\":\"4f81090f-592c-45e7-be4d-a81cce47bd0f\"},{\"content\":{\"blockPath\":[\"SwarmSystem/Record\"],\"channel\":[9,6,3],\"dimensions\":[9,9,3],\"domain\":\"SwarmSystem/Record\",\"lineColor\":\"#fe330a\",\"parentID\":5326,\"plots\":[],\"port\":9,\"sid\":[\"\"],\"signalID\":5932,\"signalName\":\"packed_tw\"},\"type\":\"RecordBlkView.Signal\",\"uuid\":\"5f8cc476-d9af-4c5e-9f21-bb7a03ef4d34\"},{\"content\":{\"blockPath\":[\"SwarmSystem/Record\"],\"channel\":[1,7,3],\"dimensions\":[9,9,3],\"domain\":\"SwarmSystem/Record\",\"lineColor\":\"#22b573\",\"parentID\":5326,\"plots\":[],\"port\":9,\"sid\":[\"\"],\"signalID\":5933,\"signalName\":\"packed_tw\"},\"type\":\"RecordBlkView.Signal\",\"uuid\":\"1933d563-f847-4ce5-bf14-abd8ee747945\"},{\"content\":{\"blockPath\":[\"SwarmSystem/Record\"],\"channel\":[2,7,3],\"dimensions\":[9,9,3],\"domain\":\"SwarmSystem/Record\",\"lineColor\":\"#0072bd\",\"parentID\":5326,\"plots\":[],\"port\":9,\"sid\":[\"\"],\"signalID\":5934,\"signalName\":\"packed_tw\"},\"type\":\"RecordBlkView.Signal\",\"uuid\":\"35eecad7-01d1-439c-9fd5-651f57443606\"},{\"content\":{\"blockPath\":[\"SwarmSystem/Record\"],\"channel\":[3,7,3],\"dimensions\":[9,9,3],\"domain\":\"SwarmSystem/Record\",\"lineColor\":\"#d95319\",\"parentID\":5326,\"plots\":[],\"port\":9,\"sid\":[\"\"],\"signalID\":5935,\"signalName\":\"packed_tw\"},\"type\":\"RecordBlkView.Signal\",\"uuid\":\"2382285d-d9f0-476e-8dcb-3003e06fb020\"},{\"content\":{\"blockPath\":[\"SwarmSystem/Record\"],\"channel\":[4,7,3],\"dimensions\":[9,9,3],\"domain\":\"SwarmSystem/Record\",\"lineColor\":\"#edb120\",\"parentID\":5326,\"plots\":[],\"port\":9,\"sid\":[\"\"],\"signalID\":5936,\"signalName\":\"packed_tw\"},\"type\":\"RecordBlkView.Signal\",\"uuid\":\"96ca900e-5afe-4c80-a74a-ffcc175baf0a\"},{\"content\":{\"blockPath\":[\"SwarmSystem/Record\"],\"channel\":[5,7,3],\"dimensions\":[9,9,3],\"domain\":\"SwarmSystem/Record\",\"lineColor\":\"#7e2f8e\",\"parentID\":5326,\"plots\":[],\"port\":9,\"sid\":[\"\"],\"signalID\":5937,\"signalName\":\"packed_tw\"},\"type\":\"RecordBlkView.Signal\",\"uuid\":\"56b4506e-745b-4f71-ae58-e73b44b26cfa\"},{\"content\":{\"blockPath\":[\"SwarmSystem/Record\"],\"channel\":[6,7,3],\"dimensions\":[9,9,3],\"domain\":\"SwarmSystem/Record\",\"lineColor\":\"#77ac30\",\"parentID\":5326,\"plots\":[],\"port\":9,\"sid\":[\"\"],\"signalID\":5938,\"signalName\":\"packed_tw\"},\"type\":\"RecordBlkView.Signal\",\"uuid\":\"279b3e00-ebc3-4a7a-b88e-87948fc7742a\"},{\"content\":{\"blockPath\":[\"SwarmSystem/Record\"],\"channel\":[7,7,3],\"dimensions\":[9,9,3],\"domain\":\"SwarmSystem/Record\",\"lineColor\":\"#4dbeee\",\"parentID\":5326,\"plots\":[],\"port\":9,\"sid\":[\"\"],\"signalID\":5939,\"signalName\":\"packed_tw\"},\"type\":\"RecordBlkView.Signal\",\"uuid\":\"7e35b6dd-51b6-4306-a589-b0f1a5869d4d\"},{\"content\":{\"blockPath\":[\"SwarmSystem/Record\"],\"channel\":[8,7,3],\"dimensions\":[9,9,3],\"domain\":\"SwarmSystem/Record\",\"lineColor\":\"#a2142f\",\"parentID\":5326,\"plots\":[],\"port\":9,\"sid\":[\"\"],\"signalID\":5940,\"signalName\":\"packed_tw\"},\"type\":\"RecordBlkView.Signal\",\"uuid\":\"7089ac8d-6b55-4184-9aef-3d0e05385dff\"},{\"content\":{\"blockPath\":[\"SwarmSystem/Record\"],\"channel\":[9,7,3],\"dimensions\":[9,9,3],\"domain\":\"SwarmSystem/Record\",\"lineColor\":\"#139fff\",\"parentID\":5326,\"plots\":[],\"port\":9,\"sid\":[\"\"],\"signalID\":5941,\"signalName\":\"packed_tw\"},\"type\":\"RecordBlkView.Signal\",\"uuid\":\"70138a80-9868-4c16-a97b-5ebad36b5e59\"},{\"content\":{\"blockPath\":[\"SwarmSystem/Record\"],\"channel\":[1,8,3],\"dimensions\":[9,9,3],\"domain\":\"SwarmSystem/Record\",\"lineColor\":\"#ff6929\",\"parentID\":5326,\"plots\":[],\"port\":9,\"sid\":[\"\"],\"signalID\":5942,\"signalName\":\"packed_tw\"},\"type\":\"RecordBlkView.Signal\",\"uuid\":\"96a1565b-bf07-4083-b7e2-dac2433cddca\"},{\"content\":{\"blockPath\":[\"SwarmSystem/Record\"],\"channel\":[2,8,3],\"dimensions\":[9,9,3],\"domain\":\"SwarmSystem/Record\",\"lineColor\":\"#b746ff\",\"parentID\":5326,\"plots\":[],\"port\":9,\"sid\":[\"\"],\"signalID\":5943,\"signalName\":\"packed_tw\"},\"type\":\"RecordBlkView.Signal\",\"uuid\":\"f456031f-d1d9-40fe-a52a-45344f90b72c\"},{\"content\":{\"blockPath\":[\"SwarmSystem/Record\"],\"channel\":[3,8,3],\"dimensions\":[9,9,3],\"domain\":\"SwarmSystem/Record\",\"lineColor\":\"#64d413\",\"parentID\":5326,\"plots\":[],\"port\":9,\"sid\":[\"\"],\"signalID\":5944,\"signalName\":\"packed_tw\"},\"type\":\"RecordBlkView.Signal\",\"uuid\":\"4ec27c7c-6dfb-4175-bc26-2973fa74d293\"},{\"content\":{\"blockPath\":[\"SwarmSystem/Record\"],\"channel\":[4,8,3],\"dimensions\":[9,9,3],\"domain\":\"SwarmSystem/Record\",\"lineColor\":\"#ff13a6\",\"parentID\":5326,\"plots\":[],\"port\":9,\"sid\":[\"\"],\"signalID\":5945,\"signalName\":\"packed_tw\"},\"type\":\"RecordBlkView.Signal\",\"uuid\":\"056aee87-a9aa-4f55-99b6-dc5ddf732552\"},{\"content\":{\"blockPath\":[\"SwarmSystem/Record\"],\"channel\":[5,8,3],\"dimensions\":[9,9,3],\"domain\":\"SwarmSystem/Record\",\"lineColor\":\"#fe330a\",\"parentID\":5326,\"plots\":[],\"port\":9,\"sid\":[\"\"],\"signalID\":5946,\"signalName\":\"packed_tw\"},\"type\":\"RecordBlkView.Signal\",\"uuid\":\"24719f4f-971b-4004-a868-c5d024c471fc\"},{\"content\":{\"blockPath\":[\"SwarmSystem/Record\"],\"channel\":[6,8,3],\"dimensions\":[9,9,3],\"domain\":\"SwarmSystem/Record\",\"lineColor\":\"#22b573\",\"parentID\":5326,\"plots\":[],\"port\":9,\"sid\":[\"\"],\"signalID\":5947,\"signalName\":\"packed_tw\"},\"type\":\"RecordBlkView.Signal\",\"uuid\":\"23cd30f4-973d-4b41-8960-36afc0fd2039\"},{\"content\":{\"blockPath\":[\"SwarmSystem/Record\"],\"channel\":[7,8,3],\"dimensions\":[9,9,3],\"domain\":\"SwarmSystem/Record\",\"lineColor\":\"#0072bd\",\"parentID\":5326,\"plots\":[],\"port\":9,\"sid\":[\"\"],\"signalID\":5948,\"signalName\":\"packed_tw\"},\"type\":\"RecordBlkView.Signal\",\"uuid\":\"9bb7d7ea-0848-424f-a0e3-921e217d9822\"},{\"content\":{\"blockPath\":[\"SwarmSystem/Record\"],\"channel\":[8,8,3],\"dimensions\":[9,9,3],\"domain\":\"SwarmSystem/Record\",\"lineColor\":\"#d95319\",\"parentID\":5326,\"plots\":[],\"port\":9,\"sid\":[\"\"],\"signalID\":5949,\"signalName\":\"packed_tw\"},\"type\":\"RecordBlkView.Signal\",\"uuid\":\"0d710afb-8f8e-4efe-bce7-0612ee3026c0\"},{\"content\":{\"blockPath\":[\"SwarmSystem/Record\"],\"channel\":[9,8,3],\"dimensions\":[9,9,3],\"domain\":\"SwarmSystem/Record\",\"lineColor\":\"#edb120\",\"parentID\":5326,\"plots\":[],\"port\":9,\"sid\":[\"\"],\"signalID\":5950,\"signalName\":\"packed_tw\"},\"type\":\"RecordBlkView.Signal\",\"uuid\":\"e6222227-238e-46f8-9bc0-fb93268f9ff2\"},{\"content\":{\"blockPath\":[\"SwarmSystem/Record\"],\"channel\":[1,9,3],\"dimensions\":[9,9,3],\"domain\":\"SwarmSystem/Record\",\"lineColor\":\"#7e2f8e\",\"parentID\":5326,\"plots\":[],\"port\":9,\"sid\":[\"\"],\"signalID\":5951,\"signalName\":\"packed_tw\"},\"type\":\"RecordBlkView.Signal\",\"uuid\":\"aa2b40c7-c9c2-4bbb-b590-0d8976a8bd7e\"},{\"content\":{\"blockPath\":[\"SwarmSystem/Record\"],\"channel\":[2,9,3],\"dimensions\":[9,9,3],\"domain\":\"SwarmSystem/Record\",\"lineColor\":\"#77ac30\",\"parentID\":5326,\"plots\":[],\"port\":9,\"sid\":[\"\"],\"signalID\":5952,\"signalName\":\"packed_tw\"},\"type\":\"RecordBlkView.Signal\",\"uuid\":\"1e95f249-b927-423d-a123-aa5a0ea44fc6\"},{\"content\":{\"blockPath\":[\"SwarmSystem/Record\"],\"channel\":[3,9,3],\"dimensions\":[9,9,3],\"domain\":\"SwarmSystem/Record\",\"lineColor\":\"#4dbeee\",\"parentID\":5326,\"plots\":[],\"port\":9,\"sid\":[\"\"],\"signalID\":5953,\"signalName\":\"packed_tw\"},\"type\":\"RecordBlkView.Signal\",\"uuid\":\"c068b22f-6793-43b6-9eb5-e65cbdaaf251\"},{\"content\":{\"blockPath\":[\"SwarmSystem/Record\"],\"channel\":[4,9,3],\"dimensions\":[9,9,3],\"domain\":\"SwarmSystem/Record\",\"lineColor\":\"#a2142f\",\"parentID\":5326,\"plots\":[],\"port\":9,\"sid\":[\"\"],\"signalID\":5954,\"signalName\":\"packed_tw\"},\"type\":\"RecordBlkView.Signal\",\"uuid\":\"5327e3cd-e7f8-4ffb-82a7-cbf250beff71\"},{\"content\":{\"blockPath\":[\"SwarmSystem/Record\"],\"channel\":[5,9,3],\"dimensions\":[9,9,3],\"domain\":\"SwarmSystem/Record\",\"lineColor\":\"#139fff\",\"parentID\":5326,\"plots\":[],\"port\":9,\"sid\":[\"\"],\"signalID\":5955,\"signalName\":\"packed_tw\"},\"type\":\"RecordBlkView.Signal\",\"uuid\":\"eb702cf1-b461-477e-a682-e9a3fd80c972\"},{\"content\":{\"blockPath\":[\"SwarmSystem/Record\"],\"channel\":[6,9,3],\"dimensions\":[9,9,3],\"domain\":\"SwarmSystem/Record\",\"lineColor\":\"#ff6929\",\"parentID\":5326,\"plots\":[],\"port\":9,\"sid\":[\"\"],\"signalID\":5956,\"signalName\":\"packed_tw\"},\"type\":\"RecordBlkView.Signal\",\"uuid\":\"27dba464-e54b-4128-82b1-2ff76222c4fa\"},{\"content\":{\"blockPath\":[\"SwarmSystem/Record\"],\"channel\":[7,9,3],\"dimensions\":[9,9,3],\"domain\":\"SwarmSystem/Record\",\"lineColor\":\"#b746ff\",\"parentID\":5326,\"plots\":[],\"port\":9,\"sid\":[\"\"],\"signalID\":5957,\"signalName\":\"packed_tw\"},\"type\":\"RecordBlkView.Signal\",\"uuid\":\"875b11e2-d967-4f15-8bdf-10426b185a6d\"},{\"content\":{\"blockPath\":[\"SwarmSystem/Record\"],\"channel\":[8,9,3],\"dimensions\":[9,9,3],\"domain\":\"SwarmSystem/Record\",\"lineColor\":\"#64d413\",\"parentID\":5326,\"plots\":[],\"port\":9,\"sid\":[\"\"],\"signalID\":5958,\"signalName\":\"packed_tw\"},\"type\":\"RecordBlkView.Signal\",\"uuid\":\"1c9882b9-a7b3-45fb-8fed-90bb0054523c\"},{\"content\":{\"blockPath\":[\"SwarmSystem/Record\"],\"channel\":[9,9,3],\"dimensions\":[9,9,3],\"domain\":\"SwarmSystem/Record\",\"lineColor\":\"#ff13a6\",\"parentID\":5326,\"plots\":[],\"port\":9,\"sid\":[\"\"],\"signalID\":5959,\"signalName\":\"packed_tw\"},\"type\":\"RecordBlkView.Signal\",\"uuid\":\"cba884c4-9507-4f2f-9df1-1fe8fd29cede\"}]},\"type\":\"RecordBlkView.InputSignals\",\"uuid\":\"21c407a8-1a28-46e4-9f24-eac3cb031d30\"}],\"packageUris\":[\"http://schema.mathworks.com/mf0/streamout_blocks/R2020a\"],\"version\":\"1.0\"}"  VisualizationBindings="{\"sparklinesplugin\":{\"info\":[{\"bindingParametersList\":[],\"subplotID\":1}]}}"
  Reshape : Reshape  OutputDimensionality=Customize  OutputDimensions=[3,3]
  Scope{,1..2,6} (4 alike) : Scope
  SwarmModel : MATLAB Function  TreatAsAtomicUnit=on
  Trajectory Attitude : Scope  NumInputPorts=3
  Trajectory Position : Scope  NumInputPorts=2
  Trajectory Velocity : Scope  NumInputPorts=2
  X Servo Profile : Scope  NumInputPorts=3
  Y Servo Profile : Scope  NumInputPorts=2
  Zero-Order Hold{,1..4} (5 alike) : ZeroOrderHold  SampleTime=dt
  wires:
  SwarmModel/1(dxdt) -> DroneState/1
  Clock/1 -> Zero-Order Hold/1  "time"
  MATLAB Function4/1(x_r) -> Multiport Selector/1, Full-Pose Controller/1(x_r)
  MATLAB Function4/2(R_r) -> MATLAB Function2/1(R), Full-Pose Controller/2(R_r)
  Multiport Selector/1 -> Trajectory Position/1  "Desired Position"
  Multiport Selector1/1 -> 6DoF Animation/1, Trajectory Position/2  "Drone Position"
  Multiport Selector1/2 -> Trajectory Velocity/2  "Drone Velocity"
  Multiport Selector/2 -> Trajectory Velocity/1  "Desired Velocity"
  Multiport Selector2/1 -> Prop1 Profile/1  "Prop Speed"
  SwarmModel/2(dzdt) -> InternalState/1
  Control Allocation/1(Tf_d) -> MATLAB Function/1(Tf_d)
  Control Allocation/2(eta_xd) -> MATLAB Function/2(eta_xd)
  Control Allocation/3(eta_yd) -> MATLAB Function/3(eta_yd)
  MATLAB Function/1(z_d) -> Zero-Order Hold4/1, Actuator Compensator/2(z_d), MATLAB Function5/1(zo), Multiport Selector5/1, Multiport Selector9/1, Multiport Selector3/1  "z_d"
  DroneState/1 -> Zero-Order Hold2/1, SwarmModel/1(x), Multiport Selector1/1
  InternalState/1 -> SwarmModel/2(z), Zero-Order Hold1/1, Matrix Multiply/2  "z"
  Multiport Selector6/1 -> Scope/1  "u_t"
  Multiport Selector7/1 -> Scope6/1  "u_tau"
  MATLAB Function1/1(eulers) -> 6DoF Animation/2, Trajectory Attitude/3  "R"
  Multiport Selector1/3 -> Reshape/1
  Reshape/1 -> MATLAB Function1/1(R)
  MATLAB Function2/1(eulers) -> Trajectory Attitude/1  "R_r"
  Full-Pose Controller/2(R_d) -> MATLAB Function3/1(R)
  MATLAB Function3/1(eulers) -> Trajectory Attitude/2  "R_d"
  Constant/1 -> Matrix Multiply/1
  MATLAB Function6/1(vec) -> Command Profile/3  "u"
  Multiport Selector3/1 -> Prop1 Profile/2  "Desired Prop Speed"
  Multiport Selector8/1 -> X Servo Profile/1  "State"
  Multiport Selector9/1 -> X Servo Profile/2  "Desired Cmd"
  Multiport Selector5/1 -> Y Servo Profile/2  "Desired Cmd"
  Multiport Selector4/1 -> Y Servo Profile/1  "State"
  Matrix Multiply/1 -> MATLAB Function6/1(zo), Multiport Selector4/1, Multiport Selector8/1, Multiport Selector2/1
  Zero-Order Hold/1 -> Record/6, MATLAB Function4/1(t)  "time"
  Actuator Compensator/1(z_dc) -> Multiport Selector10/1, SwarmModel/3(z_d)
  Multiport Selector10/1 -> X Servo Profile/3  "Over-drived"
  Zero-Order Hold1/1 -> Actuator Compensator/1(z), Zero-Order Hold3/1, Control Allocation/2(z)
  Zero-Order Hold2/1 -> Full-Pose Controller/3(x)
  Multiport Selector11/1 -> MATLAB Function7/1(u)  "Prop Speed"
  Multiport Selector12/1 -> MATLAB Function7/2(u_d)  "Prop Speed"
  Multiport Selector14/1 -> MATLAB Function8/2(u_d)  "Prop Speed"
  Multiport Selector13/1 -> MATLAB Function8/1(u)  "Prop Speed"
  Full-Pose Controller/1(u_d) -> Multiport Selector12/1, Multiport Selector14/1, Command Profile/1, Control Allocation/1(u_d), Multiport Selector6/1, Multiport Selector7/1  "u_d"
  MATLAB Function5/1(vec) -> Multiport Selector13/1, Multiport Selector11/1, Command Profile/2  "sat(u_d)"
  MATLAB Function7/2(error) -> Error Profile/1  "Position Error"
  MATLAB Function8/2(error) -> Error Profile/2  "Attitude Error"
  MATLAB Function7/1(alignment) -> Alignment Profile/1  "Position Alignment"
  MATLAB Function8/1(alignment) -> Alignment Profile/2  "Attitude Alignment"
  Control Allocation/4(N_esp) -> Record/3  "Z_esp"
  Control Allocation/5(incre) -> Record/4, Scope1/1  "increment"
  Control Allocation/6(packed_meta) -> Record/5  "bounds"
  Zero-Order Hold3/1 -> Record/1  "z"
  Zero-Order Hold4/1 -> Record/2  "z_d"
  Control Allocation/10(validness) -> Scope2/1
  Control Allocation/7(packed_detail) -> Record/7  "raw"
  Control Allocation/11(sat_order) -> Record/8  "sat_order"
  Control Allocation/8(packed_tw) -> Record/9  "packed_tw"
  Control Allocation/9(packed_intersections) -> Record/10  "packed_intersections"
